simulink library "ebs_rebuild_generic_std"  (R2016a)
settings: Solver=VariableStepAuto  StartTime=0.0  StopTime=10.0  RelTol=1e-3
undefined symbols (not defined in the file): sMP
(part 1 of 2)
settings Model: Creator=CAB  LastModifiedBy=CAB
settings GRTTargetCC: GeneratePreprocessorConditionals=Use local settings

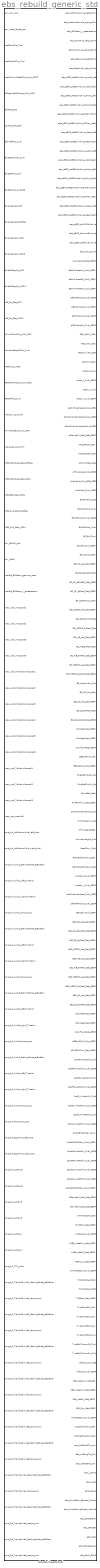
== system ebs_rebuild_generic_std ==
  ebs_rebuild_generic_std : Subsystem  mask{s1=sMP.ctrl.ebs.settings_iMode, s2=sMP.ctrl.ebs.settings_dt, initCmd='Parameters_ebs_rebuild_generic_std_sf', p1=sMP.ctrl.ebs.dim_xAxis_zSoll, p2=sMP.ctrl.ebs.veh.ABS_L1o, p3=sMP.ctrl.ebs.veh.ABS_L1v, p4=sMP.ctrl.ebs.veh.ABS_L2o, p5=sMP.ctrl.ebs.veh.ABS_L2v, p6=sMP.ctrl.ebs.veh.ABS_MinusB, p7=sMP.ctrl.ebs.veh.ABS_PlusB, p8=sMP.ctrl.ebs.veh.ABS_PlusOB, p9=sMP.ctrl.ebs.veh.ABS_THe, p10=sMP.ctrl.ebs.veh.ABS_TPulHold, p11=sMP.ctrl.ebs.veh.ABS_TPulOpen, p12=sMP.ctrl.ebs.veh.ABS_vMin_kmh, p13=sMP.ctrl.ebs.veh.flagTrailerABS, p14=sMP.ctrl.ebs.veh.rdynFA, p15=sMP.ctrl.ebs.veh.rdynRA, p16=sMP.ctrl.ebs.veh.rdynTA, p17=sMP.ctrl.ebs.veh.stepSize, p18=sMP.ctrl.ebs.ALB_dpMin_bar, p19=sMP.ctrl.ebs.ALB_mRA_Max_kg, p20=sMP.ctrl.ebs.ALB_mRA_Min_kg, p21=sMP.ctrl.ebs.ALB_p1Ref_bar, p22=sMP.ctrl.ebs.ALB_p2Max_bar, p23=sMP.ctrl.ebs.ALB_p2Min_bar, p24=sMP.ctrl.ebs.EBI_mueMax, p25=sMP.ctrl.ebs.EBI_vMin_kmh, p26=sMP.ctrl.ebs.flag_ABS, p27=sMP.ctrl.ebs.flag_DownhillDriveTest, p28=sMP.ctrl.ebs.flag_EBI, p29=sMP.ctrl.ebs.flag_SlopeCompActive, p30=sMP.ctrl.ebs.mec_iDiffAxle, p31=sMP.ctrl.ebs.Recuperation_end, p32=sMP.ctrl.ebs.Recuperation_initial, p33=sMP.ctrl.ebs.out.aAutoOpMd_Stat_SBSP, p34=sMP.ctrl.ebs.out.aBrkAirPressAA_Cval_SBSP, p35=sMP.ctrl.ebs.out.aBrkAirPressFA_Cval_SBSP, p36=sMP.ctrl.ebs.out.aBrkAirPressRA_Cval_SBSP, p37=sMP.ctrl.ebs.out.aBrkPdlPosn3_Cval_SBSP, p38=sMP.ctrl.ebs.out.aBrkTempFA_Cval_SBSP, p39=sMP.ctrl.ebs.out.aBrkTempIA_Cval_SBSP, p40=sMP.ctrl.ebs.out.aBrkTempRA_Cval_SBSP, p41=sMP.ctrl.ebs.out.ABS_Actv2_Stat, p42=sMP.ctrl.ebs.out.ABS_Actv_Stat, p43=sMP.ctrl.ebs.out.ABS_FullyOp_Stat, p44=sMP.ctrl.ebs.out.ABS_Trlr_Stat, p45=sMP.ctrl.ebs.out.Accel_X_Cval, p46=sMP.ctrl.ebs.out.Accel_X_Cval_SBSP, p47=sMP.ctrl.ebs.out.Accel_Y_Cval, p48=sMP.ctrl.ebs.out.Accel_Y_Cval_SBSP, p49=sMP.ctrl.ebs.in.ActlEmotTrq_Cval, p50=sMP.ctrl.ebs.in.ActlEngPctTrq_Cval, p51=sMP.ctrl.ebs.in.ActlMaxAvlRetPctTrq_Cval_CPC3, p52=sMP.ctrl.ebs.out.AddInfoVehSped_Cval_SBSP, p53=sMP.ctrl.ebs.out.aGroCmbVehWeight_Cval_SBSP, p54=sMP.ctrl.ebs.out.aGroCmbVehWeightConf_SBSP, p55=sMP.ctrl.ebs.in.aSbspVehBrkForce_Cmd_SDS, p56=sMP.ctrl.ebs.out.aStandstill_Dtct_Stat_SBSP, p57=sMP.ctrl.ebs.out.ATC_BrkCtrl_Stat, p58=sMP.ctrl.ebs.out.ATC_EngCtrl_Stat, p59=sMP.ctrl.ebs.out.ATC_InfoSgl_Stat, p60=sMP.ctrl.ebs.out.aTCV_Press_Cval_SBSP, p61=sMP.ctrl.ebs.out.aVehSpd_Cval_E2E_SBSP, p62=sMP.ctrl.ebs.out.aVehSpd_Cval_SBSP, p63=sMP.ctrl.ebs.out.BlockTend_Stat, p64=sMP.ctrl.ebs.out.BrkPdlPosn3_Cval, p65=sMP.ctrl.ebs.out.BrkPdlPosn3_Cval_SBSP, p66=sMP.ctrl.ebs.out.BrkPdlPosn_Cval, p67=sMP.ctrl.ebs.in.BrkPress_Rq, p68=sMP.ctrl.ebs.out.BS_Brk_Cval, p69=sMP.ctrl.ebs.out.BS_Brk_Cval_SBSP, p70=sMP.ctrl.ebs.out.BS_CS_Acc_Stat, p71=sMP.ctrl.ebs.out.BS_CS_Acc_Stat_SBSP, p72=sMP.ctrl.ebs.out.BS_CS_RqPerf2_Stat, p73=sMP.ctrl.ebs.out.BS_CS_RqPerf2_Stat_SBSP, p74=sMP.ctrl.ebs.out.BS_CS_RqPerf_Stat_SBSP, p75=sMP.ctrl.ebs.out.BS_CSCPC_Acc_Stat, p76=sMP.ctrl.ebs.out.BS_CSCPC_Acc_Stat_SBSP, p77=sMP.ctrl.ebs.out.BS_CSCPC_Intf_Stat, p78=sMP.ctrl.ebs.out.BS_CSCPC_RqPerf_Stat, p79=sMP.ctrl.ebs.out.BS_HB_Acc_Stat_SBSP, p80=sMP.ctrl.ebs.out.BS_HB_RqPerf_Stat, p81=sMP.ctrl.ebs.out.BS_HB_RqPerf_Stat_SBSP, p82=sMP.ctrl.ebs.out.BS_HBCPC_Acc_Stat_SBSP, p83=sMP.ctrl.ebs.out.BS_HBCPC_RqPerf_Stat_SBSP, p84=sMP.ctrl.ebs.out.BS_RoadIncln_Cval, p85=sMP.ctrl.ebs.out.BS_SS_Acc_Stat, p86=sMP.ctrl.ebs.out.BS_SS_Acc_Stat_SBSP, p87=sMP.ctrl.ebs.out.BS_SS_RqPerf_Stat, p88=sMP.ctrl.ebs.out.BS_SS_RqPerf_Stat_SBSP, p89=sMP.ctrl.ebs.in.Clutch_Stat_CPC, p90=sMP.ctrl.ebs.out.ConfLatAccel_SBSP, p91=sMP.ctrl.ebs.out.ConfLgtAccel_SBSP, p92=sMP.ctrl.ebs.out.ConfYawRate_SBSP, p93=sMP.ctrl.ebs.in.drv_BrkPdl_pos, p94=sMP.ctrl.ebs.in.drv_PkBrk, p95=sMP.ctrl.ebs.out.ebs_ActlEmotTrq_Nm, p96=sMP.ctrl.ebs.out.ebs_ActlEngTrq_Nm, p97=sMP.ctrl.ebs.out.ebs_ActlRetTrq_Nm, p98=sMP.ctrl.ebs.out.ebs_AdditionalAxle_left_pDmd, p99=sMP.ctrl.ebs.out.ebs_AdditionalAxle_right_pDmd, p100=sMP.ctrl.ebs.out.EBS_BrkSw2_Rq, p101=sMP.ctrl.ebs.out.EBS_BrkSw2_Rq_SBSP, p102=sMP.ctrl.ebs.out.ebs_ESCsens_y_acceleration, p103=sMP.ctrl.ebs.out.ebs_FrontAxle_left_pDmd, p104=sMP.ctrl.ebs.out.ebs_FrontAxle_right_pDmd, p105=sMP.ctrl.ebs.out.ebs_i_Emot, p106=sMP.ctrl.ebs.out.ebs_i_Ret, p107=sMP.ctrl.ebs.out.ebs_kappa, p108=sMP.ctrl.ebs.out.ebs_RearAxle_left_pDmd, p109=sMP.ctrl.ebs.out.ebs_RearAxle_right_pDmd, p110=sMP.ctrl.ebs.out.ebs_sBSP_stABSInValve_Addl_Left, p111=sMP.ctrl.ebs.out.ebs_sBSP_stABSInValve_Addl_Right, p112=sMP.ctrl.ebs.out.ebs_sBSP_stABSInValve_Front_Left, p113=sMP.ctrl.ebs.out.ebs_sBSP_stABSInValve_Front_Right, p114=sMP.ctrl.ebs.out.ebs_sBSP_stABSInValve_RCMax_Front, p115=sMP.ctrl.ebs.out.ebs_sBSP_stABSInValve_RCMax_Rear, p116=sMP.ctrl.ebs.out.ebs_sBSP_stABSInValve_Rear_Left, p117=sMP.ctrl.ebs.out.ebs_sBSP_stABSInValve_Rear_Right, p118=sMP.ctrl.ebs.out.ebs_sBSP_stABSOutValve_Addl_Left, p119=sMP.ctrl.ebs.out.ebs_sBSP_stABSOutValve_Addl_Right, p120=sMP.ctrl.ebs.out.ebs_sBSP_stABSOutValve_Front_Left, p121=sMP.ctrl.ebs.out.ebs_sBSP_stABSOutValve_Front_Right, p122=sMP.ctrl.ebs.out.ebs_sBSP_stABSOutValve_RCMax_Front, p123=sMP.ctrl.ebs.out.ebs_sBSP_stABSOutValve_RCMax_Rear, p124=sMP.ctrl.ebs.out.ebs_sBSP_stABSOutValve_Rear_Left, p125=sMP.ctrl.ebs.out.ebs_sBSP_stABSOutValve_Rear_Right, p126=sMP.ctrl.ebs.out.ebs_sBSP_stAPCVBuValve, p127=sMP.ctrl.ebs.out.ebs_sBSP_stAxmoBuValve, p128=sMP.ctrl.ebs.out.ebs_sBSP_stCMaxBuValve, p129=sMP.ctrl.ebs.out.ebs_SumBrakingForces_Trailer, p130=sMP.ctrl.ebs.out.ebs_SumBrakingForces_Vehicle, p131=sMP.ctrl.ebs.out.ebs_TCV_pDmd, p132=sMP.ctrl.ebs.out.ebs_zReqBrake, p133=sMP.ctrl.ebs.out.ebs_zReqEB, p134=sMP.ctrl.ebs.out.ebs_zRet, p135=sMP.ctrl.ebs.out.ebs_zSlopeComp, p136=sMP.ctrl.ebs.out.ebs_zSoll_BWG, p137=sMP.ctrl.ebs.in.EdrvRefTrq_Cval, p138=sMP.ctrl.ebs.in.EngPctTrqActl_Cval, p139=sMP.ctrl.ebs.in.EngRefTrq_Cval, p140=sMP.ctrl.ebs.out.EngRetTrqMax_Rq, p141=sMP.ctrl.ebs.out.EngRetTrqMin_Rq, p142=sMP.ctrl.ebs.in.EngRPM_Cval_CPC3, p143=sMP.ctrl.ebs.in.env_curv_pm, p144=sMP.ctrl.ebs.in.env_road_slope_pct, p145=sMP.ctrl.ebs.in.ExtAccel_Rq_CPC5ce, p146=sMP.ctrl.ebs.in.ExtAccel_Rq_CPC, p147=sMP.ctrl.ebs.in.ExtAccel_Rq_VRDU3, p148=sMP.ctrl.ebs.in.ExtAccel_Rq_VRDU, p149=sMP.ctrl.ebs.in.ExtBrkStat_Rq_CPC, p150=sMP.ctrl.ebs.in.ExtBrkStat_Rq_VRDU, p151=sMP.ctrl.ebs.out.FoundBrk_Stat, p152=sMP.ctrl.ebs.out.FullBrkAllow_Stat_SBSP, p153=sMP.ctrl.ebs.out.GroCmbVehWeight_Cval, p154=sMP.ctrl.ebs.in.HB_Rq_Stat_CPC, p155=sMP.ctrl.ebs.in.HB_Rq_Stat_VRDU, p156=sMP.ctrl.ebs.out.HillHolderAvl_Stat, p157=sMP.ctrl.ebs.in.mec3d_ESCsens_gamma_rate, p158=sMP.ctrl.ebs.in.mec3d_ESCsens_y_acceleration, p159=sMP.ctrl.ebs.in.mec_veh_AxleLoad1, p160=sMP.ctrl.ebs.in.mec_veh_AxleLoad2, p161=sMP.ctrl.ebs.in.mec_veh_AxleLoad3, p162=sMP.ctrl.ebs.in.mec_veh_AxleLoad4, p163=sMP.ctrl.ebs.in.mec_veh_Trailer02AxleLoad1, p164=sMP.ctrl.ebs.in.mec_veh_Trailer02AxleLoad2, p165=sMP.ctrl.ebs.in.mec_veh_Trailer02AxleLoad3, p166=sMP.ctrl.ebs.in.mec_veh_Trailer02AxleLoad4, p167=sMP.ctrl.ebs.in.mec_veh_Trailer02AxleLoad5, p168=sMP.ctrl.ebs.in.mec_veh_Trailer02AxleLoad6, p169=sMP.ctrl.ebs.in.mec_veh_TrailerAxleLoad1, p170=sMP.ctrl.ebs.in.mec_veh_TrailerAxleLoad2, p171=sMP.ctrl.ebs.in.mec_veh_TrailerAxleLoad3, p172=sMP.ctrl.ebs.in.mec_veh_transVel, p173=sMP.ctrl.ebs.in.MinAvlEmotTrq_Cval_CPC, p174=sMP.ctrl.ebs.in.NomFrictEngPctTrq_Cval, p175=sMP.ctrl.ebs.out.NrTrlr_Stat_SBSP, p176=sMP.ctrl.ebs.in.PkBrk_Rq_VRDU, p177=sMP.ctrl.ebs.in.pne_brk_AdditionalAxle_left_pAct, p178=sMP.ctrl.ebs.in.pne_brk_AdditionalAxle_right_pAct, p179=sMP.ctrl.ebs.in.pne_brk_Axle1_BrakingForce_at8p5bar, p180=sMP.ctrl.ebs.in.pne_brk_Axle1_left_Tinterior, p181=sMP.ctrl.ebs.in.pne_brk_Axle1_right_Tinterior, p182=sMP.ctrl.ebs.in.pne_brk_Axle1_torque_sns, p183=sMP.ctrl.ebs.in.pne_brk_Axle2_BrakingForce_at8p5bar, p184=sMP.ctrl.ebs.in.pne_brk_Axle2_left_Tinterior, p185=sMP.ctrl.ebs.in.pne_brk_Axle2_right_Tinterior, p186=sMP.ctrl.ebs.in.pne_brk_Axle2_torque_sns, p187=sMP.ctrl.ebs.in.pne_brk_Axle3_BrakingForce_at8p5bar, p188=sMP.ctrl.ebs.in.pne_brk_Axle3_left_Tinterior, p189=sMP.ctrl.ebs.in.pne_brk_Axle3_right_Tinterior, p190=sMP.ctrl.ebs.in.pne_brk_Axle3_torque_sns, p191=sMP.ctrl.ebs.in.pne_brk_Axle4_BrakingForce_at8p5bar, p192=sMP.ctrl.ebs.in.pne_brk_Axle4_left_Tinterior, p193=sMP.ctrl.ebs.in.pne_brk_Axle4_right_Tinterior, p194=sMP.ctrl.ebs.in.pne_brk_Axle4_torque_sns, p195=sMP.ctrl.ebs.in.pne_brk_FrontAxle_pAct, p196=sMP.ctrl.ebs.in.pne_brk_RearAxle_left_pAct, p197=sMP.ctrl.ebs.in.pne_brk_RearAxle_right_pAct, p198=sMP.ctrl.ebs.in.pne_brk_rotVel_al, p199=sMP.ctrl.ebs.in.pne_brk_rotVel_ar, p200=sMP.ctrl.ebs.in.pne_brk_rotVel_fl, p201=sMP.ctrl.ebs.in.pne_brk_rotVel_fr, p202=sMP.ctrl.ebs.in.pne_brk_rotVel_rl, p203=sMP.ctrl.ebs.in.pne_brk_rotVel_rr, p204=sMP.ctrl.ebs.in.pne_brk_TCV_pAct, p205=sMP.ctrl.ebs.in.pne_brk_Trailer02Axle1_BrakingForce_at8p5bar, p206=sMP.ctrl.ebs.in.pne_brk_Trailer02Axle1_torque_sns, p207=sMP.ctrl.ebs.in.pne_brk_Trailer02Axle2_BrakingForce_at8p5bar, p208=sMP.ctrl.ebs.in.pne_brk_Trailer02Axle2_torque_sns, p209=sMP.ctrl.ebs.in.pne_brk_Trailer02Axle3_BrakingForce_at8p5bar, p210=sMP.ctrl.ebs.in.pne_brk_Trailer02Axle3_torque_sns, p211=sMP.ctrl.ebs.in.pne_brk_Trailer02Axle4_BrakingForce_at8p5bar, p212=sMP.ctrl.ebs.in.pne_brk_Trailer02Axle4_torque_sns, p213=sMP.ctrl.ebs.in.pne_brk_Trailer02Axle5_BrakingForce_at8p5bar, p214=sMP.ctrl.ebs.in.pne_brk_Trailer02Axle5_torque_sns, p215=sMP.ctrl.ebs.in.pne_brk_Trailer02Axle6_BrakingForce_at8p5bar, p216=sMP.ctrl.ebs.in.pne_brk_Trailer02Axle6_torque_sns, p217=sMP.ctrl.ebs.in.pne_brk_TrailerAxle1_BrakingForce_at8p5bar, p218=sMP.ctrl.ebs.in.pne_brk_TrailerAxle1_torque_sns, p219=sMP.ctrl.ebs.in.pne_brk_TrailerAxle2_BrakingForce_at8p5bar, p220=sMP.ctrl.ebs.in.pne_brk_TrailerAxle2_torque_sns, p221=sMP.ctrl.ebs.in.pne_brk_TrailerAxle3_BrakingForce_at8p5bar, p222=sMP.ctrl.ebs.in.pne_brk_TrailerAxle3_torque_sns, p223=sMP.ctrl.ebs.out.PwrVehWeight_Cval, p224=sMP.ctrl.ebs.in.RetPctTrqActl2_Cval_CPC3, p225=sMP.ctrl.ebs.in.RetRefTrq_Cval, p226=sMP.ctrl.ebs.out.RoadCurv_Cval, p227=sMP.ctrl.ebs.out.ROP_BrkCtrlActv2_Stat, p228=sMP.ctrl.ebs.out.ROP_EngCtrlActv2_Stat, p229=sMP.ctrl.ebs.out.sAccel_X_Cval_SBSP, p230=sMP.ctrl.ebs.out.sAccel_Y_Cval_SBSP, p231=sMP.ctrl.ebs.out.sAddInfoVehSped_Cval_SBSP, p232=sMP.ctrl.ebs.out.sBrkPdlPosn3_Cval_SBSP, p233=sMP.ctrl.ebs.out.sBS_Brk_Cval_SBSP, p234=sMP.ctrl.ebs.out.sBS_CS_Acc_Stat_SBSP, p235=sMP.ctrl.ebs.out.sBS_CS_RqPerf2_Stat_SBSP, p236=sMP.ctrl.ebs.out.sBS_CS_RqPerf_Stat_SBSP, p237=sMP.ctrl.ebs.out.sBS_CSCPC_Acc_Stat_SBSP, p238=sMP.ctrl.ebs.out.sBS_HB_Acc_Stat_SBSP, p239=sMP.ctrl.ebs.out.sBS_HB_RqPerf_Stat_SBSP, p240=sMP.ctrl.ebs.out.sBS_HBCPC_Acc_Stat_SBSP, p241=sMP.ctrl.ebs.out.sBS_HBCPC_RqPerf_Stat_SBSP, p242=sMP.ctrl.ebs.out.sBS_SS_Acc_Stat_SBSP, p243=sMP.ctrl.ebs.out.sBS_SS_RqPerf_Stat_SBSP, p244=sMP.ctrl.ebs.out.sConfLatAccel_SBSP, p245=sMP.ctrl.ebs.out.sConfLgtAccel_SBSP, p246=sMP.ctrl.ebs.out.sConfYawRate_SBSP, p247=sMP.ctrl.ebs.out.sEBS_BrkSw2_Rq_SBSP, p248=sMP.ctrl.ebs.out.sFullBrkAllow_Stat_SBSP, p249=sMP.ctrl.ebs.out.SpdFtAxleLtWhl_Cval, p250=sMP.ctrl.ebs.out.SpdFtAxleLtWhl_Cval_SBSP, p251=sMP.ctrl.ebs.out.SpdFtAxleRtWhl_Cval, p252=sMP.ctrl.ebs.out.SpdFtAxleRtWhl_Cval_SBSP, p253=sMP.ctrl.ebs.out.SpdR_AxleLtWhl_Cval, p254=sMP.ctrl.ebs.out.SpdR_AxleLtWhl_Cval_SBSP, p255=sMP.ctrl.ebs.out.SpdR_AxleRtWhl_Cval, p256=sMP.ctrl.ebs.out.SpdR_AxleRtWhl_Cval_SBSP, p257=sMP.ctrl.ebs.out.SrcAdrBrkCtrlDev_Cval, p258=sMP.ctrl.ebs.out.SrcAdrBrkCtrlDev_Cval_SBSP, p259=sMP.ctrl.ebs.out.sSpdFtAxleLtWhl_Cval_SBSP, p260=sMP.ctrl.ebs.out.sSpdFtAxleRtWhl_Cval_SBSP, p261=sMP.ctrl.ebs.out.sSpdR_AxleLtWhl_Cval_SBSP, p262=sMP.ctrl.ebs.out.sSpdR_AxleRtWhl_Cval_SBSP, p263=sMP.ctrl.ebs.out.sSrcAdrBrkCtrlDev_Cval_SBSP, p264=sMP.ctrl.ebs.out.sStandstill_Dtct_Stat_SBSP, p265=sMP.ctrl.ebs.out.Standstill_Dtct_Stat_SBSP, p266=sMP.ctrl.ebs.out.sTrlrAbsOper_Stat, p267=sMP.ctrl.ebs.out.sTrlrEstm_Stat_SBSP, p268=sMP.ctrl.ebs.out.sVehSpd_Cval_SBSP, p269=sMP.ctrl.ebs.out.sXBR_AccelLim_Stat_SBSP, p270=sMP.ctrl.ebs.out.sXBR_ActCtrl_Stat_SBSP, p271=sMP.ctrl.ebs.out.sXBR_Sys_Stat_SBSP, p272=sMP.ctrl.ebs.out.sYawRateCorr_Cval_SBSP, p273=sMP.ctrl.ebs.out.TrctrAbsOper_Stat, p274=sMP.ctrl.ebs.out.TrlrAbsOper_Stat, p275=sMP.ctrl.ebs.out.TrlrEstm_Stat_SBSP, p276=sMP.ctrl.ebs.in.TrqConv_Cval_PT, p277=sMP.ctrl.ebs.in.TxInShaftSpd_Cval_CPC, p278=sMP.ctrl.ebs.out.TyreCorrLtFA_Cval, p279=sMP.ctrl.ebs.out.TyreCorrLtRA_Cval, p280=sMP.ctrl.ebs.out.TyreCorrRtFA_Cval, p281=sMP.ctrl.ebs.out.TyreCorrRtRA_Cval, p282=sMP.ctrl.ebs.out.TyreRollCircumFA_Cval, p283=sMP.ctrl.ebs.out.TyreRollCircumRA_Cval, p284=sMP.ctrl.ebs.in.VehSpd1_Cval_Trlr, p285=sMP.ctrl.ebs.out.VehSpd_Cval_BS, p286=sMP.ctrl.ebs.out.VehSpd_Cval_SBSP, p287=sMP.ctrl.ebs.out.XBR_AccelLim_Stat_BS, p288=sMP.ctrl.ebs.out.XBR_AccelLim_Stat_SBSP, p289=sMP.ctrl.ebs.out.XBR_ActCtrl_Stat_SBSP, p290=sMP.ctrl.ebs.in.XBR_CtrlMode_Stat_CPC5ce, p291=sMP.ctrl.ebs.in.XBR_CtrlMode_Stat_VRDU, p292=sMP.ctrl.ebs.in.XBR_EBI_Stat_VRDU, p293=sMP.ctrl.ebs.in.XBR_Prio_Stat_CPC5ce, p294=sMP.ctrl.ebs.in.XBR_Prio_Stat_VRDU, p295=sMP.ctrl.ebs.out.XBR_Sys_Stat_SBSP, p296=sMP.ctrl.ebs.out.YawRateCorr_Cval_SBSP, p297=sMP.ctrl.ebs.out.YC_BrkCtrlActv2_Stat, p298=sMP.ctrl.ebs.out.YC_EngCtrlActv2_Stat, p299=sMP.ctrl.ebs.zSoll_dx_xAxis_nom, p300=sMP.ctrl.ebs.zSoll_dx_yAxis_nom, p301=sMP.ctrl.ebs.veh.axleLoadTrailer02_kg, p302=sMP.ctrl.ebs.veh.axleLoadTrailer_kg, p303=sMP.ctrl.ebs.veh.axleLoadVehicle_kg, p304=sMP.ctrl.ebs.veh.brkCircuit, p305=sMP.ctrl.ebs.veh.flagTrailer02ControlActive, p306=sMP.ctrl.ebs.veh.flagTrailerControlActive, p307=sMP.ctrl.ebs.veh.pAppCyl_Tractor, p308=sMP.ctrl.ebs.veh.pAppCyl_Trailer, p309=sMP.ctrl.ebs.veh.pAppCyl_Trailer02, p310=sMP.ctrl.ebs.veh.rdynTrailer02, p311=sMP.ctrl.ebs.veh.speedSensorPosnVeh}
      mask prompts: s1 "Solver Type: settings_iMode [-]"; s2 "Solver Step Size: settings_dt [s]"; initCmd "Initialization command"; p1 "Dimension x-Axis zSoll-Curve [max. 40] export=true name=dim_xAxis_zSoll prio=1 dataSetName=ebs_dummy dataClassType=main dataClassName=main  unit='-' description='Dimension x-Axis zSoll-Curve': BWG.dim_xAxis_zSoll [-]"; p2 "Velocity Offset L1o (km/h) export=true name=ABS_L1o prio=1 dataSetName=veh_dummy dataClassType=veh dataClassName=veh unit='km/h' description='Velocity Offset L1o (km/h)': eBS_veh_Param.ABS_L1o [-]"; p3 "Speed Fraction for Threshold Speed 1 (0.01%) export=true name=ABS_L1v prio=1 dataSetName=veh_dummy dataClassType=veh dataClassName=veh unit='' description='Speed Fraction for Threshold Speed 1 (0.01%)': eBS_veh_Param.ABS_L1v [-]"; p4 "Velocity Offset L2o (km/h) export=true name=ABS_L2o prio=1 dataSetName=veh_dummy dataClassType=veh dataClassName=veh unit='km/h' description='Velocity Offset L2o (km/h)': eBS_veh_Param.ABS_L2o [-]"; p5 "Speed Fraction for Threshold Speed 2 (0.01%) export=true name=ABS_L2v prio=1 dataSetName=veh_dummy dataClassType=veh dataClassName=veh unit='' description='Speed Fraction for Threshold Speed 2 (0.01%)': eBS_veh_Param.ABS_L2v [-]"; p6 "Decceleration Threshold in [g] export=true name=ABS_MinusB prio=1 dataSetName=veh_dummy dataClassType=veh dataClassName=veh unit='' description='Decceleration Threshold in [g]': eBS_veh_Param.ABS_MinusB [-]"; p7 "Acceleration Threshold in [g] export=true name=ABS_PlusB prio=1 dataSetName=veh_dummy dataClassType=veh dataClassName=veh unit='' description='Decceleration Threshold in [g]': eBS_veh_Param.ABS_PlusB [-]"; p8 "Upper Acceleration Threshold in [g] export=true name=ABS_PlusOB prio=1 dataSetName=veh_dummy dataClassType=veh dataClassName=veh unit='' description='Upper Acceleration Threshold in [g]': eBS_veh_Param.ABS_PlusOB [-]"; p9 "Holding Time [ms] export=true name=ABS_THe prio=1 dataSetName=veh_dummy dataClassType=veh dataClassName=veh unit='ms' description='Holding Time [ms]': eBS_veh_Param.ABS_THe [-]"; p10 "Holding Time for Pulsating Pressure Build-Up [ms] export=true name=ABS_TPulHold prio=1 dataSetName=veh_dummy dataClassType=veh dataClassName=veh unit='ms' description='Holding Time for Pulsating Pressure Build-Up [ms]': eBS_veh_Param.ABS_TPulHold [-]"; p11 "Opening Time for Pulsating Pressure Build-Up [ms] export=true name=ABS_TPulOpen prio=1 dataSetName=veh_dummy dataClassType=veh dataClassName=veh unit='ms' description='Opening Time for Pulsating Pressure Build-Up [ms]': eBS_veh_Param.ABS_TPulOpen [-]"; p12 "Minimum Velocity for ABS Activity [km/h] export=true name=ABS_vMin_kmh prio=1 dataSetName=veh_dummy dataClassType=veh dataClassName=veh unit='km/h' description='Minimum Velocity for ABS Activity [km/h]': eBS_veh_Param.ABS_vMin_kmh [-]"; p13 "Trailer ABS Config (0 - none, 1- ABS, 2 - EBS (incl. ABS)), used in pneAux export=true name=flagTrailerABS prio=1 dataSetName=veh_dummy dataClassType=veh dataClassName=veh unit='-' description='Trailer ABS Config (0 - none, 1- ABS, 2 - EBS (incl. ABS))': eBS_veh_Param.flagTrailerABS [-]"; p14 "Dyn. Wheel Radius Front Axle [mm] export=true name=rdynFA prio=1 dataSetName=veh_dummy dataClassType=veh dataClassName=veh unit='mm' description='Dyn. Wheel Radius Front Axle [mm]': eBS_veh_Param.rdynFA [-]"; p15 "Dyn. Wheel Radius Rear Axle [mm] export=true name=rdynRA prio=1 dataSetName=veh_dummy dataClassType=veh dataClassName=veh unit='mm' description='Dyn. Wheel Radius Rear Axle [mm]': eBS_veh_Param.rdynRA [-]"; p16 "Dyn. Wheel Radius Trailer Axle [mm] export=true name=rdynTA prio=1 dataSetName=veh_dummy dataClassType=veh dataClassName=veh unit='mm' description='Dyn. Wheel Radius Trailer Axle [mm]': eBS_veh_Param.rdynTA [-]"; p17 "step Size [s] export=true name=stepSize prio=1 dataSetName=veh_dummy dataClassType=veh dataClassName=veh unit='s' description=' step size [s]': eBS_veh_Param.stepSize [s]"; p18 "ALB Linear Pressure Range p2/p1->1:1 export=true name=ALB_dpMin_bar prio=1 dataSetName=ebs_dummy dataClassType=main dataClassName=main unit=bar description='ALB Linear Pressure Range p2/p1->1:1': eBSParam.ALB_dpMin_bar [-]"; p19 "ALB Maximal Rear Axle Load for p2Max [kg] export=true name=ALB_mRA_Max_kg prio=1 dataSetName=ebs_dummy dataClassType=main dataClassName=main unit=kg description='ALB Maximal Rear Axle Load for p2Max [kg]': eBSParam.ALB_mRA_Max_kg [-]"; p20 "ALB Minimal Rear Axle Load for p2Min [kg] export=true name=ALB_mRA_Min_kg prio=1 dataSetName=ebs_dummy dataClassType=main dataClassName=main unit=kg description='ALB Minimal Rear Axle Load for p2Min [kg]': eBSParam.ALB_mRA_Min_kg [-]"; p21 "ALB Reference Inlet Pressure p1 [bar] export=true name=ALB_p1Ref_bar prio=1 dataSetName=ebs_dummy dataClassType=main dataClassName=main unit=bar description='ALB Reference Inlet Pressure p1 [bar]': eBSParam.ALB_p1Ref_bar [-]"; p22 "ALB Maximum Pressure at mRA_Max_kg [bar] export=true name=ALB_p2Max_bar prio=1 dataSetName=ebs_dummy dataClassType=main dataClassName=main unit=bar description='ALB Maximum Pressure at mRA_Max_kg [bar]': eBSParam.ALB_p2Max_bar [-]"; p23 "ALB Minimum Pressure at mRA_Min [bar] export=true name=ALB_p2Min_bar prio=1 dataSetName=ebs_dummy dataClassType=main dataClassName=main unit=bar description='ALB Minimum Pressure at mRA_Min [bar]': eBSParam.ALB_p2Min_bar [-]"; p24 "Maximum Friction Coefficient Rear Axle export=true name=EBI_mueMax prio=1 dataSetName=ebs_dummy dataClassType=main dataClassName=main unit='-' description='Maximum Friction Coefficient Rear Axle': eBSParam.EBI_mueMax [-]"; p25 "Minum Initial Velocity [km/h] (eBIActive>EBI_vMin_kmh) export=true name=EBI_vMin_kmh prio=1 dataSetName=ebs_dummy dataClassType=main dataClassName=main unit='km/h' description='Minum Initial Velocity [km/h] (eBIActive>EBI_vMin_kmh)': eBSParam.EBI_vMin_kmh [-]"; p26 "Vehicle with ABS-Brake System [0-false,1-true] export=true name=flag_ABS prio=1 dataSetName=ebs_dummy dataClassType=main dataClassName=main unit='-' description='Vehicle with ABS-Brake System [0-false,1-true]': eBSParam.flag_ABS [-]"; p27 "Flag Downhill Drive Test [0-false,1-true] export=true name=flag_DownhillDriveTest prio=1 dataSetName=ebs_dummy dataClassType=main dataClassName=main unit='-' description='Flag Downhill Drive Test [0-false,1-true]': eBSParam.flag_DownhillDriveTest [-]"; p28 "Endurance Brake Integration (EBI) [0-no EBI,1-EBI, base deceleration of 2% by service brake, 2- EBI 100%, 3 - prior endurance brake activation, 4 - EBI Bus mode] export=true name=flag_EBI prio=1 dataSetName=ebs_dummy dataClassType=main dataClassName=main unit='-' description='Endurance Brake Integration (EBI) [0-no EBI,1-EBI, base deceleration of 2% by service brake, 2- EBI 100%, 3 - prior endurance brake activation, 4 - EBI Bus mode]': eBSParam.flag_EBI [-]"; p29 "Slope Compensation Active [0 - false,1 - true] export=true name=flag_SlopeCompActive prio=1 dataSetName=ebs_dummy dataClassType=main dataClassName=main unit='-' description='Slope Compensation Active [0 - false,1 - true]': eBSParam.flag_SlopeCompActive [-]"; p30 "Transmission Ratio EMot - Axle [-] export=true name=mec_iDiffAxle prio=1 dataSetName=ebs_dummy dataClassType=main dataClassName=main unit='' description='Transmission Ratio EMot - Axle [-]': eBSParam.mec_iDiffAxle [-]"; p31 "Recuperation value for full brake pedal actuation [Nm] export=true name=Recuperation_end prio=1 dataSetName=ebs_dummy dataClassType=main dataClassName=main unit=kg description='Recuperation value for inital brake pedal actuation [Nm] ': eBSParam.Recuperation_end [-]"; p32 "Recuperation value for inital brake pedal actuation [Nm] export=true name=Recuperation_initial prio=1 dataSetName=ebs_dummy dataClassType=main dataClassName=main unit=kg description='Recuperation value for inital brake pedal actuation [Nm] ': eBSParam.Recuperation_initial [-]"; p33 "aAutoOpMd_Stat_SBSP export=true name=aAutoOpMd_Stat_SBSP prio=1 dataSetName=std dataClassType=initIO dataClassName=initIO unit='-' description='aAutoOpMd_Stat_SBSP': IO_EBS_InputSignals.aAutoOpMd_Stat_SBSP_0 [-]"; p34 "aBrkAirPressAA_Cval_SBSP export=true name=aBrkAirPressAA_Cval_SBSP prio=1 dataSetName=std dataClassType=initIO dataClassName=initIO unit='kPa' description='aBrkAirPressAA_Cval_SBSP': IO_EBS_InputSignals.aBrkAirPressAA_Cval_SBSP_0 [-]"; p35 "aBrkAirPressFA_Cval_SBSP export=true name=aBrkAirPressFA_Cval_SBSP prio=1 dataSetName=std dataClassType=initIO dataClassName=initIO unit='kPa' description='aBrkAirPressFA_Cval_SBSP': IO_EBS_InputSignals.aBrkAirPressFA_Cval_SBSP_0 [-]"; p36 "aBrkAirPressRA_Cval_SBSP export=true name=aBrkAirPressRA_Cval_SBSP prio=1 dataSetName=std dataClassType=initIO dataClassName=initIO unit='kPa' description='aBrkAirPressRA_Cval_SBSP': IO_EBS_InputSignals.aBrkAirPressRA_Cval_SBSP_0 [-]"; p37 "aBrkPdlPosn3_Cval_SBSP export=true name=aBrkPdlPosn3_Cval_SBSP prio=1 dataSetName=std dataClassType=initIO dataClassName=initIO unit='%' description='aBrkPdlPosn3_Cval_SBSP': IO_EBS_InputSignals.aBrkPdlPosn3_Cval_SBSP_0 [-]"; p38 "aBrkTempFA_Cval_SBSP export=true name=aBrkTempFA_Cval_SBSP prio=1 dataSetName=std dataClassType=initIO dataClassName=initIO unit='degC' description='aBrkTempFA_Cval_SBSP': IO_EBS_InputSignals.aBrkTempFA_Cval_SBSP_0 [-]"; p39 "aBrkTempIA_Cval_SBSP export=true name=aBrkTempIA_Cval_SBSP prio=1 dataSetName=std dataClassType=initIO dataClassName=initIO unit='degC' description='aBrkTempIA_Cval_SBSP': IO_EBS_InputSignals.aBrkTempIA_Cval_SBSP_0 [-]"; p40 "aBrkTempRA_Cval_SBSP export=true name=aBrkTempRA_Cval_SBSP prio=1 dataSetName=std dataClassType=initIO dataClassName=initIO unit='degC' description='aBrkTempRA_Cval_SBSP': IO_EBS_InputSignals.aBrkTempRA_Cval_SBSP_0 [-]"; p41 "ABS_Actv2_Stat export=true name=ABS_Actv2_Stat prio=1 dataSetName=std dataClassType=initIO dataClassName=initIO unit='-' description='ABS_Actv2_Stat': IO_EBS_InputSignals.ABS_Actv2_Stat_0 [-]"; p42 "ABS_Actv_Stat export=true name=ABS_Actv_Stat prio=1 dataSetName=std dataClassType=initIO dataClassName=initIO unit='-' description='ABS_Actv_Stat': IO_EBS_InputSignals.ABS_Actv_Stat_0 [-]"; p43 "ABS_FullyOp_Stat export=true name=ABS_FullyOp_Stat prio=1 dataSetName=std dataClassType=initIO dataClassName=initIO unit='-' description='ABS_FullyOp_Stat': IO_EBS_InputSignals.ABS_FullyOp_Stat_0 [-]"; p44 "ABS_Trlr_Stat export=true name=ABS_Trlr_Stat prio=1 dataSetName=std dataClassType=initIO dataClassName=initIO unit='-' description='ABS_Trlr_Stat': IO_EBS_InputSignals.ABS_Trlr_Stat_0 [-]"; p45 "ABS61449S_E_LongitudAcc, 255 SNA; export=true name=Accel_X_Cval prio=1 dataSetName=std dataClassType=initIO dataClassName=initIO unit='m/s^2' description='ABS61449S_E_LongitudAcc, 255 SNA;': IO_EBS_InputSignals.Accel_X_Cval_0 [-]"; p46 "ABS61449S_E_LongitudAcc, 255 SNA; export=true name=Accel_X_Cval_SBSP prio=1 dataSetName=std dataClassType=initIO dataClassName=initIO unit='m/s^2' description='ABS61449S_E_LongitudAcc, 255 SNA;': IO_EBS_InputSignals.Accel_X_Cval_SBSP_0 [-]"; p47 "Accel_Y_Cval export=true name=Accel_Y_Cval prio=1 dataSetName=std dataClassType=initIO dataClassName=initIO unit=m/s^2 description='Accel_Y_Cval': IO_EBS_InputSignals.Accel_Y_Cval_0 [-]"; p48 "Accel_Y_Cval_SBSP export=true name=Accel_Y_Cval_SBSP prio=1 dataSetName=std dataClassType=initIO dataClassName=initIO unit=m/s^2 description='Accel_Y_Cval_SBSP': IO_EBS_InputSignals.Accel_Y_Cval_SBSP_0 [-]"; p49 "ActlEmotTrq_Cval (init) export=true name=ActlEmotTrq_Cval prio=1 dataSetName=std dataClassType=initIO dataClassName=initIO unit='-' description='ActlEmotTrq_Cval (init)': IO_EBS_InputSignals.ActlEmotTrq_Cval_0 [-]"; p50 "ActlEngPctTrq_Cval export=true name=ActlEngPctTrq_Cval prio=1 dataSetName=std dataClassType=initIO dataClassName=initIO unit='-' description='ActlEngPctTrq_Cval': IO_EBS_InputSignals.ActlEngPctTrq_Cval_0 [-]"; p51 "ActlMaxAvlRetPctTrq_Cval_CPC3 export=true name=ActlMaxAvlRetPctTrq_Cval_CPC3 prio=1 dataSetName=std dataClassType=initIO dataClassName=initIO unit='-' description='ActlMaxAvlRetPctTrq_Cval_CPC3': IO_EBS_InputSignals.ActlMaxAvlRetPctTrq_Cval_CPC3_0 [-]"; p52 "AddInfoVehSped_Cval_SBSP (init) export=true name=AddInfoVehSped_Cval_SBSP prio=1 dataSetName=std dataClassType=initIO dataClassName=initIO unit='' description='AddInfoVehSped_Cval_SBSP': IO_EBS_InputSignals.AddInfoVehSped_Cval_SBSP_0 [-]"; p53 "aGroCmbVehWeight_Cval_SBSP export=true name=aGroCmbVehWeight_Cval_SBSP prio=1 dataSetName=std dataClassType=initIO dataClassName=initIO unit='kg' description='aGroCmbVehWeight_Cval_SBSP': IO_EBS_InputSignals.aGroCmbVehWeight_Cval_SBSP_0 [-]"; p54 "aGroCmbVehWeightConf_SBSP export=true name=aGroCmbVehWeightConf_SBSP prio=1 dataSetName=std dataClassType=initIO dataClassName=initIO unit='%' description='Vehicle Mass estimate confidence factor': IO_EBS_InputSignals.aGroCmbVehWeightConf_SBSP_0 [-]"; p55 "aSbspVehBrkForce_Cmd_SDS export=true name=aSbspVehBrkForce_Cmd_SDS prio=1 dataSetName=std dataClassType=initIO dataClassName=initIO unit='N' description='aSbspVehBrkForce_Cmd_SDS': IO_EBS_InputSignals.aSbspVehBrkForce_Cmd_SDS_0 [-]"; p56 "aStandstill_Dtct_Stat_SBSP export=true name=aStandstill_Dtct_Stat_SBSP prio=1 dataSetName=std dataClassType=initIO dataClassName=initIO unit='-' description='Standstill detected Current state': IO_EBS_InputSignals.aStandstill_Dtct_Stat_SBSP_0 [-]"; p57 "ATC_BrkCtrl_Stat export=true name=ATC_BrkCtrl_Stat prio=1 dataSetName=std dataClassType=initIO dataClassName=initIO unit='-' description='ATC_BrkCtrl_Stat': IO_EBS_InputSignals.ATC_BrkCtrl_Stat_0 [-]"; p58 "ATC_EngCtrl_Stat export=true name=ATC_EngCtrl_Stat prio=1 dataSetName=std dataClassType=initIO dataClassName=initIO unit='-' description='ATC_EngCtrl_Stat': IO_EBS_InputSignals.ATC_EngCtrl_Stat_0 [-]"; p59 "ATC_InfoSgl_Stat export=true name=ATC_InfoSgl_Stat prio=1 dataSetName=std dataClassType=initIO dataClassName=initIO unit='-' description='ATC_InfoSgl_Stat': IO_EBS_InputSignals.ATC_InfoSgl_Stat_0 [-]"; p60 "aTCV_Press_Cval_SBSP export=true name=aTCV_Press_Cval_SBSP prio=1 dataSetName=std dataClassType=initIO dataClassName=initIO unit='kPa' description='aTCV_Press_Cval_SBSP': IO_EBS_InputSignals.aTCV_Press_Cval_SBSP_0 [-]"; p61 "aVehSpd_Cval_E2E_SBSP export=true name=aVehSpd_Cval_E2E_SBSP prio=1 dataSetName=std dataClassType=initIO dataClassName=initIO unit='km/h' description='aVehSpd_Cval_E2E_SBSP': IO_EBS_InputSignals.aVehSpd_Cval_E2E_SBSP_0 [-]"; p62 "aVehSpd_Cval_SBSP export=true name=aVehSpd_Cval_SBSP prio=1 dataSetName=std dataClassType=initIO dataClassName=initIO unit='km/h' description='Vehicle Speed Current value': IO_EBS_InputSignals.aVehSpd_Cval_SBSP_0 [-]"; p63 "BlockTend_Stat export=true name=BlockTend_Stat prio=1 dataSetName=std dataClassType=initIO dataClassName=initIO unit='-' description='BlockTend_Stat': IO_EBS_InputSignals.BlockTend_Stat_0 [-]"; p64 "Brake Pedal Position 3 Current value (an CPC3) export=true name=BrkPdlPosn3_Cval prio=1 dataSetName=std dataClassType=initIO dataClassName=initIO unit='%' description='Brake Pedal Position 3 Current value (an CPC3)': IO_EBS_InputSignals.BrkPdlPosn3_Cval_0 [-]"; p65 "Brake Pedal Position 3 Current value (an CPC3) export=true name=BrkPdlPosn3_Cval_SBSP prio=1 dataSetName=std dataClassType=initIO dataClassName=initIO unit='%' description='Brake Pedal Position 3 Current value (an CPC3) SBSP': IO_EBS_InputSignals.BrkPdlPosn3_Cval_SBSP_0 [-]"; p66 "Brake Pedal Position Current value (an CGW) export=true name=BrkPdlPosn_Cval prio=1 dataSetName=std dataClassType=initIO dataClassName=initIO unit='%' description='Brake Pedal Position Current value (an CGW)': IO_EBS_InputSignals.BrkPdlPosn_Cval_0 [-]"; p67 "BrkPress_Rq export=true name=BrkPress_Rq prio=1 dataSetName=std dataClassType=initIO dataClassName=initIO unit='-' description='BrkPress_Rq': IO_EBS_InputSignals.BrkPress_Rq_0 [-]"; p68 "Brake Current value, 254 ERR; 255 SNA; export=true name=BS_Brk_Cval prio=1 dataSetName=std dataClassType=initIO dataClassName=initIO unit='%' description='Brake Current value, 254 ERR; 255 SNA;': IO_EBS_InputSignals.BS_Brk_Cval_0 [-]"; p69 "Brake Current value, 254 ERR; 255 SNA; export=true name=BS_Brk_Cval_SBSP prio=1 dataSetName=std dataClassType=initIO dataClassName=initIO unit='%' description='Brake Current value, 254 ERR; 255 SNA; SBSP': IO_EBS_InputSignals.BS_Brk_Cval_SBSP_0 [-]"; p70 "BS_CS_Acc_Stat export=true name=BS_CS_Acc_Stat prio=1 dataSetName=std dataClassType=initIO dataClassName=initIO unit='-' description='BS_CSCPC_Acc_Stat': IO_EBS_InputSignals.BS_CS_Acc_Stat_0 [-]"; p71 "BS_CS_Acc_Stat_SBSP export=true name=BS_CS_Acc_Stat_SBSP prio=1 dataSetName=std dataClassType=initIO dataClassName=initIO unit='-' description='BS_CSCPC_Acc_Stat': IO_EBS_InputSignals.BS_CS_Acc_Stat_SBSP_0 [-]"; p72 "BS_CS_RqPerf2_Stat export=true name=BS_CS_RqPerf2_Stat prio=1 dataSetName=std dataClassType=initIO dataClassName=initIO unit='-' description='BS_CS_RqPerf2_Stat': IO_EBS_InputSignals.BS_CS_RqPerf2_Stat_0 [-]"; p73 "BS_CS_RqPerf2_Stat_SBSP export=true name=BS_CS_RqPerf2_Stat_SBSP prio=1 dataSetName=std dataClassType=initIO dataClassName=initIO unit='-' description='BS_CS_RqPerf2_Stat_SBSP': IO_EBS_InputSignals.BS_CS_RqPerf2_Stat_SBSP_0 [-]"; p74 "BS_CS_RqPerf_Stat_SBSP export=true name=BS_CS_RqPerf_Stat_SBSP prio=1 dataSetName=std dataClassType=initIO dataClassName=initIO unit='-' description='BS_CS_RqPerf_Stat_SBSP': IO_EBS_InputSignals.BS_CS_RqPerf_Stat_SBSP_0 [-]"; p75 "BS_CSCPC_Acc_Stat export=true name=BS_CSCPC_Acc_Stat prio=1 dataSetName=std dataClassType=initIO dataClassName=initIO unit='-' description='BS_CSCPC_Acc_Stat': IO_EBS_InputSignals.BS_CSCPC_Acc_Stat_0 [-]"; p76 "BS_CSCPC_Acc_Stat_SBSP export=true name=BS_CSCPC_Acc_Stat_SBSP prio=1 dataSetName=std dataClassType=initIO dataClassName=initIO unit='-' description='BS_CSCPC_Acc_Stat_SBSP': IO_EBS_InputSignals.BS_CSCPC_Acc_Stat_SBSP_0 [-]"; p77 "BS_CSCPC_Intf_Stat export=true name=BS_CSCPC_Intf_Stat prio=1 dataSetName=std dataClassType=initIO dataClassName=initIO unit='-' description='BS_CSCPC_Intf_Stat': IO_EBS_InputSignals.BS_CSCPC_Intf_Stat_0 [-]"; p78 "BS_CSCPC_RqPerf_Stat export=true name=BS_CSCPC_RqPerf_Stat prio=1 dataSetName=std dataClassType=initIO dataClassName=initIO unit='-' description='BS_CSCPC_RqPerf_Stat': IO_EBS_InputSignals.BS_CSCPC_RqPerf_Stat_0 [-]"; p79 "BS_HB_Acc_Stat_SBSP export=true name=BS_HB_Acc_Stat_SBSP prio=1 dataSetName=std dataClassType=initIO dataClassName=initIO unit='-' description='BS_HB_Acc_Stat_SBSP': IO_EBS_InputSignals.BS_HB_Acc_Stat_SBSP_0 [-]"; p80 "Brake Current value, 254 ERR; 255 SNA; export=true name=BS_HB_RqPerf_Stat prio=1 dataSetName=std dataClassType=initIO dataClassName=initIO unit='-' description='Brake Current value, 254 ERR; 255 SNA;': IO_EBS_InputSignals.BS_HB_RqPerf_Stat_0 [-]"; p81 "Brake Current value, 254 ERR; 255 SNA; export=true name=BS_HB_RqPerf_Stat_SBSP prio=1 dataSetName=std dataClassType=initIO dataClassName=initIO unit='-' description='Brake Current value, 254 ERR; 255 SNA; SBSP': IO_EBS_InputSignals.BS_HB_RqPerf_Stat_SBSP_0 [-]"; p82 "BS_HBCPC_Acc_Stat_SBSP export=true name=BS_HBCPC_Acc_Stat_SBSP prio=1 dataSetName=std dataClassType=initIO dataClassName=initIO unit='-' description='BS_HBCPC_Acc_Stat_SBSP': IO_EBS_InputSignals.BS_HBCPC_Acc_Stat_SBSP_0 [-]"; p83 "BS_HBCPC_RqPerf_Stat_SBSP export=true name=BS_HBCPC_RqPerf_Stat_SBSP prio=1 dataSetName=std dataClassType=initIO dataClassName=initIO unit='-' description='BS_HBCPC_RqPerf_Stat_SBSP': IO_EBS_InputSignals.BS_HBCPC_RqPerf_Stat_SBSP_0 [-]"; p84 "Road inclination current value (calculated), 254 ERR; 255 SNA; export=true name=BS_RoadIncln_Cval prio=1 dataSetName=std dataClassType=initIO dataClassName=initIO unit='%' description='Road inclination current value (calculated), 254 ERR; 255 SNA;': IO_EBS_InputSignals.BS_RoadIncln_Cval_0 [-]"; p85 "BS_SS_Acc_Stat export=true name=BS_SS_Acc_Stat prio=1 dataSetName=std dataClassType=initIO dataClassName=initIO unit='-' description='BS_CSCPC_Acc_Stat': IO_EBS_InputSignals.BS_SS_Acc_Stat_0 [-]"; p86 "BS_SS_Acc_Stat_SBSP export=true name=BS_SS_Acc_Stat_SBSP prio=1 dataSetName=std dataClassType=initIO dataClassName=initIO unit='-' description='BS_CSCPC_Acc_Stat': IO_EBS_InputSignals.BS_SS_Acc_Stat_SBSP_0 [-]"; p87 "BS_SS_RqPerf_Stat export=true name=BS_SS_RqPerf_Stat prio=1 dataSetName=std dataClassType=initIO dataClassName=initIO unit='-' description='BS_SS_RqPerf_Stat': IO_EBS_InputSignals.BS_SS_RqPerf_Stat_0 [-]"; p88 "BS_SS_RqPerf_Stat_SBSP export=true name=BS_SS_RqPerf_Stat_SBSP prio=1 dataSetName=std dataClassType=initIO dataClassName=initIO unit='-' description='BS_SS_RqPerf_Stat_SBSP': IO_EBS_InputSignals.BS_SS_RqPerf_Stat_SBSP_0 [-]"; p89 "Clutch_Stat_CPC (init) export=true name=Clutch_Stat_CPC prio=1 dataSetName=std dataClassType=initIO dataClassName=initIO unit='-' description='Clutch_Stat_CPC (init)': IO_EBS_InputSignals.Clutch_Stat_CPC_0 [-]"; p90 "ConfLatAccel_SBSP (init) export=true name=ConfLatAccel_SBSP prio=1 dataSetName=std dataClassType=initIO dataClassName=initIO unit='%' description='ConfLatAccel_SBSP': IO_EBS_InputSignals.ConfLatAccel_SBSP_0 [-]"; p91 "ConfLgtAccel_SBSP (init) export=true name=ConfLgtAccel_SBSP prio=1 dataSetName=std dataClassType=initIO dataClassName=initIO unit='%' description='ConfLgtAccel_SBSP': IO_EBS_InputSignals.ConfLgtAccel_SBSP_0 [-]"; p92 "ConfYawRate_SBSP (init) export=true name=ConfYawRate_SBSP prio=1 dataSetName=std dataClassType=initIO dataClassName=initIO unit='%' description='ConfYawRate_SBSP': IO_EBS_InputSignals.ConfYawRate_SBSP_0 [-]"; p93 "drv_BrkPdl_pos export=true name=drv_BrkPdl_pos prio=1 dataSetName=std dataClassType=initIO dataClassName=initIO unit='-' description='drv_BrkPdl_pos': IO_EBS_InputSignals.drv_BrkPdl_pos_0 [-]"; p94 "drv_PkBrk export=true name=drv_PkBrk prio=1 dataSetName=std dataClassType=initIO dataClassName=initIO unit='-' description='drv_PkBrk': IO_EBS_InputSignals.drv_PkBrk_0 [-]"; p95 "ebs_ActlEmotTrq_Nm export=true name=ebs_ActlEmotTrq_Nm prio=1 dataSetName=std dataClassType=initIO dataClassName=initIO unit=Nm description='ebs_ActlEmotTrq_Nm': IO_EBS_InputSignals.ebs_ActlEmotTrq_Nm_0 [-]"; p96 "ebs_ActlEngTrq_Nm export=true name=ebs_ActlEngTrq_Nm prio=1 dataSetName=std dataClassType=initIO dataClassName=initIO unit=Nm description='ebs_ActlEngTrq_Nm': IO_EBS_InputSignals.ebs_ActlEngTrq_Nm_0 [-]"; p97 "ebs_ActlRetTrq_Nm export=true name=ebs_ActlRetTrq_Nm prio=1 dataSetName=std dataClassType=initIO dataClassName=initIO unit=Nm description='ebs_ActlRetTrq_Nm': IO_EBS_InputSignals.ebs_ActlRetTrq_Nm_0 [-]"; p98 "ebs_AdditionalAxle_left_pDmd (init) export=true name=ebs_AdditionalAxle_left_pDmd prio=1 dataSetName=std dataClassType=initIO dataClassName=initIO unit='-' description='ebs_AdditionalAxle_left_pDmd': IO_EBS_InputSignals.ebs_AdditionalAxle_left_pDmd_0 [-]"; p99 "ebs_AdditionalAxle_right_pDmd (init) export=true name=ebs_AdditionalAxle_right_pDmd prio=1 dataSetName=std dataClassType=initIO dataClassName=initIO unit='-' description='ebs_AdditionalAxle_right_pDmd': IO_EBS_InputSignals.ebs_AdditionalAxle_right_pDmd_0 [-]"; p100 "EBS Brake Switch 2 Request state for DTR+, 0 NPSD; 1 PSD; 2 ERR; 3 SNA; export=true name=EBS_BrkSw2_Rq prio=1 dataSetName=std dataClassType=initIO dataClassName=initIO unit='-' description='EBS Brake Switch 2 Request state for DTR+, 0 NPSD; 1 PSD; 2 ERR; 3 SNA;': IO_EBS_InputSignals.EBS_BrkSw2_Rq_0 [-]"; p101 "EBS Brake Switch 2 Request state for DTR+, 0 NPSD; 1 PSD; 2 ERR; 3 SNA; export=true name=EBS_BrkSw2_Rq_SBSP prio=1 dataSetName=std dataClassType=initIO dataClassName=initIO unit='-' description='EBS Brake Switch 2 Request state for DTR+, 0 NPSD; 1 PSD; 2 ERR; 3 SNA;': IO_EBS_InputSignals.EBS_BrkSw2_Rq_SBSP_0 [-]"; p102 "ebs_ESCsens_y_acceleration export=true name=ebs_ESCsens_y_acceleration prio=1 dataSetName=std dataClassType=initIO dataClassName=initIO unit='m/s^2' description='ebs_ESCsens_y_acceleration': IO_EBS_InputSignals.ebs_ESCsens_y_acceleration_0 [-]"; p103 "ebs_FrontAxle_left_pDmd (init) export=true name=ebs_FrontAxle_left_pDmd prio=1 dataSetName=std dataClassType=initIO dataClassName=initIO unit='-' description='ebs_FrontAxle_left_pDmd': IO_EBS_InputSignals.ebs_FrontAxle_left_pDmd_0 [-]"; p104 "ebs_FrontAxle_right_pDmd (init) export=true name=ebs_FrontAxle_right_pDmd prio=1 dataSetName=std dataClassType=initIO dataClassName=initIO unit='-' description='ebs_FrontAxle_right_pDmd': IO_EBS_InputSignals.ebs_FrontAxle_right_pDmd_0 [-]"; p105 "ebs_i_Emot export=true name=ebs_i_Emot prio=1 dataSetName=std dataClassType=initIO dataClassName=initIO unit='-' description='ebs_i_Emot': IO_EBS_InputSignals.ebs_i_Emot_0 [-]"; p106 "ebs_i_Ret export=true name=ebs_i_Ret prio=1 dataSetName=std dataClassType=initIO dataClassName=initIO unit='-' description='ebs_i_Ret': IO_EBS_InputSignals.ebs_i_Ret_0 [-]"; p107 "ebs_kappa export=true name=ebs_kappa prio=1 dataSetName=std dataClassType=initIO dataClassName=initIO unit='-' description='ebs_kappa': IO_EBS_InputSignals.ebs_kappa_0 [-]"; p108 "ebs_RearAxle_left_pDmd (init) export=true name=ebs_RearAxle_left_pDmd prio=1 dataSetName=std dataClassType=initIO dataClassName=initIO unit='-' description='ebs_RearAxle_left_pDmd': IO_EBS_InputSignals.ebs_RearAxle_left_pDmd_0 [-]"; p109 "ebs_RearAxle_right_pDmd (init) export=true name=ebs_RearAxle_right_pDmd prio=1 dataSetName=std dataClassType=initIO dataClassName=initIO unit='-' description='ebs_RearAxle_right_pDmd': IO_EBS_InputSignals.ebs_RearAxle_right_pDmd_0 [-]"; p110 "ebs_sBSP_stABSInValve_Addl_Left export=true name=ebs_sBSP_stABSInValve_Addl_Left prio=1 dataSetName=std dataClassType=initIO dataClassName=initIO unit='-' description='ebs_sBSP_stABSInValve_Addl_Left': IO_EBS_InputSignals.ebs_sBSP_stABSInValve_Addl_Left_0 [-]"; p111 "ebs_sBSP_stABSInValve_Addl_Right export=true name=ebs_sBSP_stABSInValve_Addl_Right prio=1 dataSetName=std dataClassType=initIO dataClassName=initIO unit='-' description='ebs_sBSP_stABSInValve_Addl_Right': IO_EBS_InputSignals.ebs_sBSP_stABSInValve_Addl_Right_0 [-]"; p112 "ebs_sBSP_stABSInValve_Front_Left export=true name=ebs_sBSP_stABSInValve_Front_Left prio=1 dataSetName=std dataClassType=initIO dataClassName=initIO unit='-' description='ebs_sBSP_stABSInValve_Front_Left': IO_EBS_InputSignals.ebs_sBSP_stABSInValve_Front_Left_0 [-]"; p113 "ebs_sBSP_stABSInValve_Front_Right export=true name=ebs_sBSP_stABSInValve_Front_Right prio=1 dataSetName=std dataClassType=initIO dataClassName=initIO unit='-' description='ebs_sBSP_stABSInValve_Front_Right': IO_EBS_InputSignals.ebs_sBSP_stABSInValve_Front_Right_0 [-]"; p114 "ebs_sBSP_stABSInValve_RCMax_Front (init),   export=true name=ebs_sBSP_stABSInValve_RCMax_Front prio=1 dataSetName=std dataClassType=initIO dataClassName=initIO unit='-' description=' ': IO_EBS_InputSignals.ebs_sBSP_stABSInValve_RCMax_Front_0 [-]"; p115 "ebs_sBSP_stABSInValve_RCMax_Rear (init),   export=true name=ebs_sBSP_stABSInValve_RCMax_Rear prio=1 dataSetName=std dataClassType=initIO dataClassName=initIO unit='-' description=' ': IO_EBS_InputSignals.ebs_sBSP_stABSInValve_RCMax_Rear_0 [-]"; p116 "ebs_sBSP_stABSInValve_Rear_Left export=true name=ebs_sBSP_stABSInValve_Rear_Left prio=1 dataSetName=std dataClassType=initIO dataClassName=initIO unit='-' description='ebs_sBSP_stABSInValve_Rear_Left': IO_EBS_InputSignals.ebs_sBSP_stABSInValve_Rear_Left_0 [-]"; p117 "ebs_sBSP_stABSInValve_Rear_Right export=true name=ebs_sBSP_stABSInValve_Rear_Right prio=1 dataSetName=std dataClassType=initIO dataClassName=initIO unit='-' description='ebs_sBSP_stABSInValve_Rear_Right': IO_EBS_InputSignals.ebs_sBSP_stABSInValve_Rear_Right_0 [-]"; p118 "ebs_sBSP_stABSOutValve_Addl_Left export=true name=ebs_sBSP_stABSOutValve_Addl_Left prio=1 dataSetName=std dataClassType=initIO dataClassName=initIO unit='-' description='ebs_sBSP_stABSOutValve_Addl_Left': IO_EBS_InputSignals.ebs_sBSP_stABSOutValve_Addl_Left_0 [-]"; p119 "ebs_sBSP_stABSOutValve_Addl_Right export=true name=ebs_sBSP_stABSOutValve_Addl_Right prio=1 dataSetName=std dataClassType=initIO dataClassName=initIO unit='-' description='ebs_sBSP_stABSOutValve_Addl_Right': IO_EBS_InputSignals.ebs_sBSP_stABSOutValve_Addl_Right_0 [-]"; p120 "ebs_sBSP_stABSOutValve_Front_Left export=true name=ebs_sBSP_stABSOutValve_Front_Left prio=1 dataSetName=std dataClassType=initIO dataClassName=initIO unit='-' description='ebs_sBSP_stABSOutValve_Front_Left': IO_EBS_InputSignals.ebs_sBSP_stABSOutValve_Front_Left_0 [-]"; p121 "ebs_sBSP_stABSOutValve_Front_Right export=true name=ebs_sBSP_stABSOutValve_Front_Right prio=1 dataSetName=std dataClassType=initIO dataClassName=initIO unit='-' description='ebs_sBSP_stABSOutValve_Front_Right': IO_EBS_InputSignals.ebs_sBSP_stABSOutValve_Front_Right_0 [-]"; p122 "ebs_sBSP_stABSOutValve_RCMax_Front (init),   export=true name=ebs_sBSP_stABSOutValve_RCMax_Front prio=1 dataSetName=std dataClassType=initIO dataClassName=initIO unit='-' description=' ': IO_EBS_InputSignals.ebs_sBSP_stABSOutValve_RCMax_Front_0 [-]"; p123 "ebs_sBSP_stABSOutValve_RCMax_Rear (init),   export=true name=ebs_sBSP_stABSOutValve_RCMax_Rear prio=1 dataSetName=std dataClassType=initIO dataClassName=initIO unit='-' description=' ': IO_EBS_InputSignals.ebs_sBSP_stABSOutValve_RCMax_Rear_0 [-]"; p124 "ebs_sBSP_stABSOutValve_Rear_Left export=true name=ebs_sBSP_stABSOutValve_Rear_Left prio=1 dataSetName=std dataClassType=initIO dataClassName=initIO unit='-' description='ebs_sBSP_stABSOutValve_Rear_Left': IO_EBS_InputSignals.ebs_sBSP_stABSOutValve_Rear_Left_0 [-]"; p125 "ebs_sBSP_stABSOutValve_Rear_Right export=true name=ebs_sBSP_stABSOutValve_Rear_Right prio=1 dataSetName=std dataClassType=initIO dataClassName=initIO unit='-' description='ebs_sBSP_stABSOutValve_Rear_Right': IO_EBS_InputSignals.ebs_sBSP_stABSOutValve_Rear_Right_0 [-]"; p126 "ebs_sBSP_stAPCVBuValve export=true name=ebs_sBSP_stAPCVBuValve prio=1 dataSetName=std dataClassType=initIO dataClassName=initIO unit='-' description='ebs_sBSP_stAPCVBuValve': IO_EBS_InputSignals.ebs_sBSP_stAPCVBuValve_0 [-]"; p127 "ebs_sBSP_stAxmoBuValve export=true name=ebs_sBSP_stAxmoBuValve prio=1 dataSetName=std dataClassType=initIO dataClassName=initIO unit='-' description='ebs_sBSP_stAxmoBuValve': IO_EBS_InputSignals.ebs_sBSP_stAxmoBuValve_0 [-]"; p128 "ebs_sBSP_stCMaxBuValve export=true name=ebs_sBSP_stCMaxBuValve prio=1 dataSetName=std dataClassType=initIO dataClassName=initIO unit='-' description='ebs_sBSP_stCMaxBuValve': IO_EBS_InputSignals.ebs_sBSP_stCMaxBuValve_0 [-]"; p129 "ebs_SumBrakingForces_Trailer (init) export=true name=ebs_SumBrakingForces_Trailer prio=1 dataSetName=std dataClassType=initIO dataClassName=initIO unit='-' description='ebs_SumBrakingForces_Trailer': IO_EBS_InputSignals.ebs_SumBrakingForces_Trailer_0 [-]"; p130 "ebs_SumBrakingForces_Vehicle (init) export=true name=ebs_SumBrakingForces_Vehicle prio=1 dataSetName=std dataClassType=initIO dataClassName=initIO unit='-' description='ebs_SumBrakingForces_Vehicle': IO_EBS_InputSignals.ebs_SumBrakingForces_Vehicle_0 [-]"; p131 "ebs_TCV_pDmd (init) export=true name=ebs_TCV_pDmd prio=1 dataSetName=std dataClassType=initIO dataClassName=initIO unit='-' description='ebs_TCV_pDmd': IO_EBS_InputSignals.ebs_TCV_pDmd_0 [-]"; p132 "ebs_zReqBrake export=true name=ebs_zReqBrake prio=1 dataSetName=std dataClassType=initIO dataClassName=initIO unit='-' description='ebs_zReqBrake': IO_EBS_InputSignals.ebs_zReqBrake_0 [-]"; p133 "ebs_zReqEB export=true name=ebs_zReqEB prio=1 dataSetName=std dataClassType=initIO dataClassName=initIO unit='-' description='ebs_zReqEB': IO_EBS_InputSignals.ebs_zReqEB_0 [-]"; p134 "ebs_zRet export=true name=ebs_zRet prio=1 dataSetName=std dataClassType=initIO dataClassName=initIO unit='-' description='ebs_zRet': IO_EBS_InputSignals.ebs_zRet_0 [-]"; p135 "ebs_zSlopeComp export=true name=ebs_zSlopeComp prio=1 dataSetName=std dataClassType=initIO dataClassName=initIO unit='-' description='ebs_zSlopeComp': IO_EBS_InputSignals.ebs_zSlopeComp_0 [-]"; p136 "ebs_zSoll_BWG export=true name=ebs_zSoll_BWG prio=1 dataSetName=std dataClassType=initIO dataClassName=initIO unit='-' description='ebs_zSoll_BWG': IO_EBS_InputSignals.ebs_zSoll_BWG_0 [-]"; p137 "EdrvRefTrq_Cval (init) export=true name=EdrvRefTrq_Cval prio=1 dataSetName=std dataClassType=initIO dataClassName=initIO unit='-' description='EdrvRefTrq_Cval (init)': IO_EBS_InputSignals.EdrvRefTrq_Cval_0 [-]"; p138 "EngPctTrqActl_Cval export=true name=EngPctTrqActl_Cval prio=1 dataSetName=std dataClassType=initIO dataClassName=initIO unit='-' description='EngPctTrqActl_Cval': IO_EBS_InputSignals.EngPctTrqActl_Cval_0 [-]"; p139 "EngRefTrq_Cval export=true name=EngRefTrq_Cval prio=1 dataSetName=std dataClassType=initIO dataClassName=initIO unit='-' description='EngRefTrq_Cval': IO_EBS_InputSignals.EngRefTrq_Cval_0 [-]"; p140 "EngRetTrqMax_Rq (toCAN) export=true name=EngRetTrqMax_Rq prio=1 dataSetName=std dataClassType=initIO dataClassName=initIO unit='-' description='EngRetTrqMax_Rq (toCAN)': IO_EBS_InputSignals.EngRetTrqMax_Rq_0 [-]"; p141 "EngRetTrqMin_Rq (to CAN) export=true name=EngRetTrqMin_Rq prio=1 dataSetName=std dataClassType=initIO dataClassName=initIO unit='-' description='EngRetTrqMin_Rq (to CAN)': IO_EBS_InputSignals.EngRetTrqMin_Rq_0 [-]"; p142 "Engine RPM Current value from CPC export=true name=EngRPM_Cval_CPC3 prio=1 dataSetName=std dataClassType=initIO dataClassName=initIO unit='-' description='Engine RPM Current value from CPC': IO_EBS_InputSignals.EngRPM_Cval_CPC3_0 [-]"; p143 "curvature of road [1/m] export=true name=env_curv_pm prio=1 dataSetName=std dataClassType=initIO dataClassName=initIO unit='-' description='curvature of road [1/m]': IO_EBS_InputSignals.env_curv_pm_0 [-]"; p144 "slope of road [%] export=true name=env_road_slope_pct prio=1 dataSetName=std dataClassType=initIO dataClassName=initIO unit='-' description='slope of road [%]': IO_EBS_InputSignals.env_road_slope_pct_0 [-]"; p145 "ExtAccel_Rq_CPC5ce [m/s^2] export=true name=ExtAccel_Rq_CPC5ce prio=1 dataSetName=std dataClassType=initIO dataClassName=initIO unit='-' description='ExtAccel_Rq_CPC5ce [m/s^2]': IO_EBS_InputSignals.ExtAccel_Rq_CPC5ce_0 [-]"; p146 "ExtAccel_Rq_CPC [m/s^2] export=true name=ExtAccel_Rq_CPC prio=1 dataSetName=std dataClassType=initIO dataClassName=initIO unit='-' description='ExtAccel_Rq_CPC [m/s^2]': IO_EBS_InputSignals.ExtAccel_Rq_CPC_0 [-]"; p147 "ExtAccel_Rq_VRDU3 export=true name=ExtAccel_Rq_VRDU3 prio=1 dataSetName=std dataClassType=initIO dataClassName=initIO unit='m/s^2' description='ACC External Acceleration Demand': IO_EBS_InputSignals.ExtAccel_Rq_VRDU3_0 [-]"; p148 "ExtAccel_Rq_VRDU [m/s^2] export=true name=ExtAccel_Rq_VRDU prio=1 dataSetName=std dataClassType=initIO dataClassName=initIO unit='-' description='ExtAccel_Rq_VRDU [m/s^2]': IO_EBS_InputSignals.ExtAccel_Rq_VRDU_0 [-]"; p149 "ExtBrkStat_Rq_CPC [-] export=true name=ExtBrkStat_Rq_CPC prio=1 dataSetName=std dataClassType=initIO dataClassName=initIO unit='-' description='ExtBrkStat_Rq_CPC [-]': IO_EBS_InputSignals.ExtBrkStat_Rq_CPC_0 [-]"; p150 "ExtBrkStat_Rq_VRDU [-] export=true name=ExtBrkStat_Rq_VRDU prio=1 dataSetName=std dataClassType=initIO dataClassName=initIO unit='-' description='ExtBrkStat_Rq_VRDU [-]': IO_EBS_InputSignals.ExtBrkStat_Rq_VRDU_0 [-]"; p151 "FoundBrk_Stat service brake is:   0 --> inaktive , 1 --> aktive, 4 --> sna export=true name=FoundBrk_Stat prio=1 dataSetName=std dataClassType=initIO dataClassName=initIO unit='-' description='FoundBrk_Stat, service brake is:   0 --> inaktive , 1 --> aktive, 4 --> sna': IO_EBS_InputSignals.FoundBrk_Stat_0 [-]"; p152 "FullBrkAllow_Stat_SBSP export=true name=FullBrkAllow_Stat_SBSP prio=1 dataSetName=std dataClassType=initIO dataClassName=initIO unit='-' description='FullBrkAllow_Stat_SBSP': IO_EBS_InputSignals.FullBrkAllow_Stat_SBSP_0 [-]"; p153 "GroCmbVehWeight_Cval (init) export=true name=GroCmbVehWeight_Cval prio=1 dataSetName=std dataClassType=initIO dataClassName=initIO unit=kg description='GroCmbVehWeight_Cval': IO_EBS_InputSignals.GroCmbVehWeight_Cval_0 [-]"; p154 "HB_Rq_Stat_CPC export=true name=HB_Rq_Stat_CPC prio=1 dataSetName=std dataClassType=initIO dataClassName=initIO unit='-' description='HB_Rq_Stat_CPC': IO_EBS_InputSignals.HB_Rq_Stat_CPC_0 [-]"; p155 "HB_Rq_Stat_VRDU export=true name=HB_Rq_Stat_VRDU prio=1 dataSetName=std dataClassType=initIO dataClassName=initIO unit='-' description='HB_Rq_Stat_VRDU': IO_EBS_InputSignals.HB_Rq_Stat_VRDU_0 [-]"; p156 "Hill Holder Availability Current State, 0 HH_AVL; 1 HH_ACTV_NOT_FF; 2 HH_MF; 3 SNA; export=true name=HillHolderAvl_Stat prio=1 dataSetName=std dataClassType=initIO dataClassName=initIO unit='-' description='Hill Holder Availability Current State, 0 HH_AVL; 1 HH_ACTV_NOT_FF; 2 HH_MF; 3 SNA;': IO_EBS_InputSignals.HillHolderAvl_Stat_0 [-]"; p157 "mec3d_ESCsens_gamma_rate export=true name=mec3d_ESCsens_gamma_rate prio=1 dataSetName=std dataClassType=initIO dataClassName=initIO unit='rad/s' description='mec3d_ESCsens_gamma_rate': IO_EBS_InputSignals.mec3d_ESCsens_gamma_rate_0 [-]"; p158 "mec3d_ESCsens_y_acceleration export=true name=mec3d_ESCsens_y_acceleration prio=1 dataSetName=std dataClassType=initIO dataClassName=initIO unit='m/s^2' description='mec3d_ESCsens_y_acceleration': IO_EBS_InputSignals.mec3d_ESCsens_y_acceleration_0 [-]"; p159 "mec_veh_AxleLoad1 (init) export=true name=mec_veh_AxleLoad1 prio=1 dataSetName=std dataClassType=initIO dataClassName=initIO unit=kg description='mec_veh_AxleLoad1': IO_EBS_InputSignals.mec_veh_AxleLoad1_0 [-]"; p160 "mec_veh_AxleLoad2 (init) export=true name=mec_veh_AxleLoad2 prio=1 dataSetName=std dataClassType=initIO dataClassName=initIO unit=kg description='mec_veh_AxleLoad2': IO_EBS_InputSignals.mec_veh_AxleLoad2_0 [-]"; p161 "mec_veh_AxleLoad3 (init) export=true name=mec_veh_AxleLoad3 prio=1 dataSetName=std dataClassType=initIO dataClassName=initIO unit=kg description='mec_veh_AxleLoad3': IO_EBS_InputSignals.mec_veh_AxleLoad3_0 [-]"; p162 "mec_veh_AxleLoad4 (init) export=true name=mec_veh_AxleLoad4 prio=1 dataSetName=std dataClassType=initIO dataClassName=initIO unit=kg description='mec_veh_AxleLoad4': IO_EBS_InputSignals.mec_veh_AxleLoad4_0 [-]"; p163 "mec_veh_Trailer02AxleLoad1 (init) export=true name=mec_veh_Trailer02AxleLoad1 prio=1 dataSetName=std dataClassType=initIO dataClassName=initIO unit=kg description='mec_veh_Trailer02AxleLoad1': IO_EBS_InputSignals.mec_veh_Trailer02AxleLoad1_0 [-]"; p164 "mec_veh_Trailer02AxleLoad2 (init) export=true name=mec_veh_Trailer02AxleLoad2 prio=1 dataSetName=std dataClassType=initIO dataClassName=initIO unit=kg description='mec_veh_Trailer02AxleLoad2': IO_EBS_InputSignals.mec_veh_Trailer02AxleLoad2_0 [-]"; p165 "mec_veh_Trailer02AxleLoad3 (init) export=true name=mec_veh_Trailer02AxleLoad3 prio=1 dataSetName=std dataClassType=initIO dataClassName=initIO unit=kg description='mec_veh_Trailer02AxleLoad3': IO_EBS_InputSignals.mec_veh_Trailer02AxleLoad3_0 [-]"; p166 "mec_veh_Trailer02AxleLoad4 (init) export=true name=mec_veh_Trailer02AxleLoad4 prio=1 dataSetName=std dataClassType=initIO dataClassName=initIO unit=kg description='mec_veh_Trailer02AxleLoad4': IO_EBS_InputSignals.mec_veh_Trailer02AxleLoad4_0 [-]"; p167 "mec_veh_Trailer02AxleLoad5 (init) export=true name=mec_veh_Trailer02AxleLoad5 prio=1 dataSetName=std dataClassType=initIO dataClassName=initIO unit=kg description='mec_veh_Trailer02AxleLoad5': IO_EBS_InputSignals.mec_veh_Trailer02AxleLoad5_0 [-]"; p168 "mec_veh_Trailer02AxleLoad6 (init) export=true name=mec_veh_Trailer02AxleLoad6 prio=1 dataSetName=std dataClassType=initIO dataClassName=initIO unit=kg description='mec_veh_Trailer02AxleLoad6': IO_EBS_InputSignals.mec_veh_Trailer02AxleLoad6_0 [-]"; p169 "mec_veh_TrailerAxleLoad1 (init) export=true name=mec_veh_TrailerAxleLoad1 prio=1 dataSetName=std dataClassType=initIO dataClassName=initIO unit=kg description='mec_veh_TrailerAxleLoad1': IO_EBS_InputSignals.mec_veh_TrailerAxleLoad1_0 [-]"; p170 "mec_veh_TrailerAxleLoad2 (init) export=true name=mec_veh_TrailerAxleLoad2 prio=1 dataSetName=std dataClassType=initIO dataClassName=initIO unit=kg description='mec_veh_TrailerAxleLoad2': IO_EBS_InputSignals.mec_veh_TrailerAxleLoad2_0 [-]"; p171 "mec_veh_TrailerAxleLoad3 (init) export=true name=mec_veh_TrailerAxleLoad3 prio=1 dataSetName=std dataClassType=initIO dataClassName=initIO unit=kg description='mec_veh_TrailerAxleLoad3': IO_EBS_InputSignals.mec_veh_TrailerAxleLoad3_0 [-]"; p172 "mec_veh_transVel export=true name=mec_veh_transVel prio=1 dataSetName=std dataClassType=initIO dataClassName=initIO unit='-' description='mec_veh_transVel': IO_EBS_InputSignals.mec_veh_transVel_0 [-]"; p173 "MinAvlEmotTrq_Cval_CPC (init) export=true name=MinAvlEmotTrq_Cval_CPC prio=1 dataSetName=std dataClassType=initIO dataClassName=initIO unit='-' description='MinAvlEmotTrq_Cval_CPC (init)': IO_EBS_InputSignals.MinAvlEmotTrq_Cval_CPC_0 [-]"; p174 "NomFrictEngPctTrq_Cval export=true name=NomFrictEngPctTrq_Cval prio=1 dataSetName=std dataClassType=initIO dataClassName=initIO unit='-' description='NomFrictEngPctTrq_Cval': IO_EBS_InputSignals.NomFrictEngPctTrq_Cval_0 [-]"; p175 "NrTrlr_Stat_SBSP (init) export=true name=NrTrlr_Stat_SBSP prio=1 dataSetName=std dataClassType=initIO dataClassName=initIO unit='' description='NrTrlr_Stat_SBSP': IO_EBS_InputSignals.NrTrlr_Stat_SBSP_0 [-]"; p176 "PkBrk_Rq_VRDU export=true name=PkBrk_Rq_VRDU prio=1 dataSetName=std dataClassType=initIO dataClassName=initIO unit='-' description='PkBrk_Rq_VRDU': IO_EBS_InputSignals.PkBrk_Rq_VRDU_0 [-]"; p177 "Front axle: acting pressure export=true name=pne_brk_AdditionalAxle_left_pAct prio=1 dataSetName=std dataClassType=initIO dataClassName=initIO unit='bar' description='actual pressure Additional leftt at 2k-AXMO': IO_EBS_InputSignals.pne_brk_AdditionalAxle_left_pAct_0 [-]"; p178 "Front axle: acting pressure export=true name=pne_brk_AdditionalAxle_right_pAct prio=1 dataSetName=std dataClassType=initIO dataClassName=initIO unit='bar' description='actual pressure Additional right at 2k-AXMO': IO_EBS_InputSignals.pne_brk_AdditionalAxle_right_pAct_0 [-]"; p179 "pne_brk_Axle1_BrakingForce_at8p5bar [N] (init) export=true name=pne_brk_Axle1_BrakingForce_at8p5bar prio=1 dataSetName=std dataClassType=initIO dataClassName=initIO unit=N description='pne_brk_Axle1_BrakingForce_at8p5bar [N] (init)': IO_EBS_InputSignals.pne_brk_Axle1_BrakingForce_at8p5bar_0 [-]"; p180 "axle 1 left temperature of the friction area [degC] (init) export=true name=pne_brk_Axle1_left_Tinterior prio=1 dataSetName=std dataClassType=initIO dataClassName=initIO unit=degC description='axle 1 left inner temperature [degC] (init)': IO_EBS_InputSignals.pne_brk_Axle1_left_Tinterior_0 [-]"; p181 "axle 1 right temperature of the friction area [degC] (init) export=true name=pne_brk_Axle1_right_Tinterior prio=1 dataSetName=std dataClassType=initIO dataClassName=initIO unit=degC description='axle 1 right inner temperature [degC] (init)': IO_EBS_InputSignals.pne_brk_Axle1_right_Tinterior_0 [-]"; p182 "pne_brk_Axle1_torque_sns export=true name=pne_brk_Axle1_torque_sns prio=1 dataSetName=std dataClassType=initIO dataClassName=initIO unit='-' description='pne_brk_Axle1_torque_sns': IO_EBS_InputSignals.pne_brk_Axle1_torque_sns_0 [-]"; p183 "pne_brk_Axle2_BrakingForce_at8p5bar [N] (init) export=true name=pne_brk_Axle2_BrakingForce_at8p5bar prio=1 dataSetName=std dataClassType=initIO dataClassName=initIO unit=N description='pne_brk_Axle2_BrakingForce_at8p5bar [N] (init)': IO_EBS_InputSignals.pne_brk_Axle2_BrakingForce_at8p5bar_0 [-]"; p184 "axle 2 left temperature of the friction area [degC] (init) export=true name=pne_brk_Axle2_left_Tinterior prio=1 dataSetName=std dataClassType=initIO dataClassName=initIO unit=degC description='axle 1 left inner temperature [degC] (init)': IO_EBS_InputSignals.pne_brk_Axle2_left_Tinterior_0 [-]"; p185 "axle 2 right temperature of the friction area [degC] (init) export=true name=pne_brk_Axle2_right_Tinterior prio=1 dataSetName=std dataClassType=initIO dataClassName=initIO unit=degC description='axle 1 right inner temperature [degC] (init)': IO_EBS_InputSignals.pne_brk_Axle2_right_Tinterior_0 [-]"; p186 "pne_brk_Axle2_torque_sns export=true name=pne_brk_Axle2_torque_sns prio=1 dataSetName=std dataClassType=initIO dataClassName=initIO unit='-' description='pne_brk_Axle2_torque_sns': IO_EBS_InputSignals.pne_brk_Axle2_torque_sns_0 [-]"; p187 "pne_brk_Axle3_BrakingForce_at8p5bar [N] (init) export=true name=pne_brk_Axle3_BrakingForce_at8p5bar prio=1 dataSetName=std dataClassType=initIO dataClassName=initIO unit=N description='pne_brk_Axle3_BrakingForce_at8p5bar [N] (init)': IO_EBS_InputSignals.pne_brk_Axle3_BrakingForce_at8p5bar_0 [-]"; p188 "axle 3 left temperature of the friction area [degC] (init) export=true name=pne_brk_Axle3_left_Tinterior prio=1 dataSetName=std dataClassType=initIO dataClassName=initIO unit=degC description='axle 1 left inner temperature [degC] (init)': IO_EBS_InputSignals.pne_brk_Axle3_left_Tinterior_0 [-]"; p189 "axle 3 right temperature of the friction area [degC] (init) export=true name=pne_brk_Axle3_right_Tinterior prio=1 dataSetName=std dataClassType=initIO dataClassName=initIO unit=degC description='axle 1 right inner temperature [degC] (init)': IO_EBS_InputSignals.pne_brk_Axle3_right_Tinterior_0 [-]"; p190 "pne_brk_Axle3_torque_sns export=true name=pne_brk_Axle3_torque_sns prio=1 dataSetName=std dataClassType=initIO dataClassName=initIO unit='-' description='pne_brk_Axle3_torque_sns': IO_EBS_InputSignals.pne_brk_Axle3_torque_sns_0 [-]"; p191 "pne_brk_Axle4_BrakingForce_at8p5bar [N] (init) export=true name=pne_brk_Axle4_BrakingForce_at8p5bar prio=1 dataSetName=std dataClassType=initIO dataClassName=initIO unit=N description='pne_brk_Axle4_BrakingForce_at8p5bar [N] (init)': IO_EBS_InputSignals.pne_brk_Axle4_BrakingForce_at8p5bar_0 [-]"; p192 "axle 4 left temperature of the friction area [degC] (init) export=true name=pne_brk_Axle4_left_Tinterior prio=1 dataSetName=std dataClassType=initIO dataClassName=initIO unit=degC description='axle 1 left inner temperature [degC] (init)': IO_EBS_InputSignals.pne_brk_Axle4_left_Tinterior_0 [-]"; p193 "axle 4 right temperature of the friction area [degC] (init) export=true name=pne_brk_Axle4_right_Tinterior prio=1 dataSetName=std dataClassType=initIO dataClassName=initIO unit=degC description='axle 1 right inner temperature [degC] (init)': IO_EBS_InputSignals.pne_brk_Axle4_right_Tinterior_0 [-]"; p194 "pne_brk_Axle4_torque_sns export=true name=pne_brk_Axle4_torque_sns prio=1 dataSetName=std dataClassType=initIO dataClassName=initIO unit='-' description='pne_brk_Axle4_torque_sns': IO_EBS_InputSignals.pne_brk_Axle4_torque_sns_0 [-]"; p195 "Front axle: acting pressure export=true name=pne_brk_FrontAxle_pAct prio=1 dataSetName=std dataClassType=initIO dataClassName=initIO unit='bar' description='Front axle: acting pressure': IO_EBS_InputSignals.pne_brk_FrontAxle_pAct_0 [-]"; p196 "Rear axle left: acting pressure export=true name=pne_brk_RearAxle_left_pAct prio=1 dataSetName=std dataClassType=initIO dataClassName=initIO unit='bar' description='Rear axle left: acting pressure': IO_EBS_InputSignals.pne_brk_RearAxle_left_pAct_0 [-]"; p197 "Rear axle right: acting pressure export=true name=pne_brk_RearAxle_right_pAct prio=1 dataSetName=std dataClassType=initIO dataClassName=initIO unit='bar' description='Rear axle right: acting pressure': IO_EBS_InputSignals.pne_brk_RearAxle_right_pAct_0 [-]"; p198 "wheel speed additional left wheel export=true name=pne_brk_rotVel_al prio=1 dataSetName=std dataClassType=initIO dataClassName=initIO unit='-' description='wheel speed additional left wheel': IO_EBS_InputSignals.pne_brk_rotVel_al_0 [-]"; p199 "wheel speed additional right wheel export=true name=pne_brk_rotVel_ar prio=1 dataSetName=std dataClassType=initIO dataClassName=initIO unit='-' description='wheel speed additional right wheel': IO_EBS_InputSignals.pne_brk_rotVel_ar_0 [-]"; p200 "wheel speed front left wheel export=true name=pne_brk_rotVel_fl prio=1 dataSetName=std dataClassType=initIO dataClassName=initIO unit='-' description='wheel speed front left wheel': IO_EBS_InputSignals.pne_brk_rotVel_fl_0 [-]"; p201 "wheel speed front right wheel export=true name=pne_brk_rotVel_fr prio=1 dataSetName=std dataClassType=initIO dataClassName=initIO unit='-' description='wheel speed front right wheel': IO_EBS_InputSignals.pne_brk_rotVel_fr_0 [-]"; p202 "wheel speed rear left wheel export=true name=pne_brk_rotVel_rl prio=1 dataSetName=std dataClassType=initIO dataClassName=initIO unit='-' description='wheel speed rear left wheel': IO_EBS_InputSignals.pne_brk_rotVel_rl_0 [-]"; p203 "wheel speed rear right wheel export=true name=pne_brk_rotVel_rr prio=1 dataSetName=std dataClassType=initIO dataClassName=initIO unit='-' description='wheel speed rear right wheel': IO_EBS_InputSignals.pne_brk_rotVel_rr_0 [-]"; p204 "Front axle: acting pressure export=true name=pne_brk_TCV_pAct prio=1 dataSetName=std dataClassType=initIO dataClassName=initIO unit='bar' description='actual pressure TCV': IO_EBS_InputSignals.pne_brk_TCV_pAct_0 [-]"; p205 "pne_brk_Trailer02Axle1_BrakingForce_at8p5bar [N] (init) export=true name=pne_brk_Trailer02Axle1_BrakingForce_at8p5bar prio=1 dataSetName=std dataClassType=initIO dataClassName=initIO unit=N description='pne_brk_Trailer02Axle1_BrakingForce_at8p5bar [N] (init)': IO_EBS_InputSignals.pne_brk_Trailer02Axle1_BrakingForce_at8p5bar_0 [-]"; p206 "pne_brk_Trailer02Axle1_torque_sns (init) export=true name=pne_brk_Trailer02Axle1_torque_sns prio=1 dataSetName=std dataClassType=initIO dataClassName=initIO unit=kg description='pne_brk_Trailer02Axle1_torque_sns': IO_EBS_InputSignals.pne_brk_Trailer02Axle1_torque_sns_0 [-]"; p207 "pne_brk_Trailer02Axle2_BrakingForce_at8p5bar [N] (init) export=true name=pne_brk_Trailer02Axle2_BrakingForce_at8p5bar prio=1 dataSetName=std dataClassType=initIO dataClassName=initIO unit=N description='pne_brk_Trailer02Axle2_BrakingForce_at8p5bar [N] (init)': IO_EBS_InputSignals.pne_brk_Trailer02Axle2_BrakingForce_at8p5bar_0 [-]"; p208 "pne_brk_Trailer02Axle2_torque_sns (init) export=true name=pne_brk_Trailer02Axle2_torque_sns prio=1 dataSetName=std dataClassType=initIO dataClassName=initIO unit=kg description='pne_brk_Trailer02Axle2_torque_sns': IO_EBS_InputSignals.pne_brk_Trailer02Axle2_torque_sns_0 [-]"; p209 "pne_brk_Trailer02Axle3_BrakingForce_at8p5bar [N] (init) export=true name=pne_brk_Trailer02Axle3_BrakingForce_at8p5bar prio=1 dataSetName=std dataClassType=initIO dataClassName=initIO unit=N description='pne_brk_Trailer02Axle3_BrakingForce_at8p5bar [N] (init)': IO_EBS_InputSignals.pne_brk_Trailer02Axle3_BrakingForce_at8p5bar_0 [-]"; p210 "pne_brk_Trailer02Axle3_torque_sns (init) export=true name=pne_brk_Trailer02Axle3_torque_sns prio=1 dataSetName=std dataClassType=initIO dataClassName=initIO unit=kg description='pne_brk_Trailer02Axle3_torque_sns': IO_EBS_InputSignals.pne_brk_Trailer02Axle3_torque_sns_0 [-]"; p211 "pne_brk_Trailer02Axle4_BrakingForce_at8p5bar [N] (init) export=true name=pne_brk_Trailer02Axle4_BrakingForce_at8p5bar prio=1 dataSetName=std dataClassType=initIO dataClassName=initIO unit=N description='pne_brk_Trailer02Axle4_BrakingForce_at8p5bar [N] (init)': IO_EBS_InputSignals.pne_brk_Trailer02Axle4_BrakingForce_at8p5bar_0 [-]"; p212 "pne_brk_Trailer02Axle4_torque_sns (init) export=true name=pne_brk_Trailer02Axle4_torque_sns prio=1 dataSetName=std dataClassType=initIO dataClassName=initIO unit=kg description='pne_brk_Trailer02Axle4_torque_sns': IO_EBS_InputSignals.pne_brk_Trailer02Axle4_torque_sns_0 [-]"; p213 "pne_brk_Trailer02Axle5_BrakingForce_at8p5bar [N] (init) export=true name=pne_brk_Trailer02Axle5_BrakingForce_at8p5bar prio=1 dataSetName=std dataClassType=initIO dataClassName=initIO unit=N description='pne_brk_Trailer02Axle5_BrakingForce_at8p5bar [N] (init)': IO_EBS_InputSignals.pne_brk_Trailer02Axle5_BrakingForce_at8p5bar_0 [-]"; p214 "pne_brk_Trailer02Axle5_torque_sns (init) export=true name=pne_brk_Trailer02Axle5_torque_sns prio=1 dataSetName=std dataClassType=initIO dataClassName=initIO unit=kg description='pne_brk_Trailer02Axle5_torque_sns': IO_EBS_InputSignals.pne_brk_Trailer02Axle5_torque_sns_0 [-]"; p215 "pne_brk_Trailer02Axle6_BrakingForce_at8p5bar [N] (init) export=true name=pne_brk_Trailer02Axle6_BrakingForce_at8p5bar prio=1 dataSetName=std dataClassType=initIO dataClassName=initIO unit=N description='pne_brk_Trailer02Axle6_BrakingForce_at8p5bar [N] (init)': IO_EBS_InputSignals.pne_brk_Trailer02Axle6_BrakingForce_at8p5bar_0 [-]"; p216 "pne_brk_Trailer02Axle6_torque_sns (init) export=true name=pne_brk_Trailer02Axle6_torque_sns prio=1 dataSetName=std dataClassType=initIO dataClassName=initIO unit=kg description='pne_brk_Trailer02Axle6_torque_sns': IO_EBS_InputSignals.pne_brk_Trailer02Axle6_torque_sns_0 [-]"; p217 "pne_brk_TrailerAxle1_BrakingForce_at8p5bar [N] (init) export=true name=pne_brk_TrailerAxle1_BrakingForce_at8p5bar prio=1 dataSetName=std dataClassType=initIO dataClassName=initIO unit=N description='pne_brk_TrailerAxle1_BrakingForce_at8p5bar [N] (init)': IO_EBS_InputSignals.pne_brk_TrailerAxle1_BrakingForce_at8p5bar_0 [-]"; p218 "pne_brk_TrailerAxle1_torque_sns export=true name=pne_brk_TrailerAxle1_torque_sns prio=1 dataSetName=std dataClassType=initIO dataClassName=initIO unit='-' description='pne_brk_TrailerAxle1_torque_sns': IO_EBS_InputSignals.pne_brk_TrailerAxle1_torque_sns_0 [-]"; p219 "pne_brk_TrailerAxle2_BrakingForce_at8p5bar [N] (init) export=true name=pne_brk_TrailerAxle2_BrakingForce_at8p5bar prio=1 dataSetName=std dataClassType=initIO dataClassName=initIO unit=N description='pne_brk_TrailerAxle2_BrakingForce_at8p5bar [N] (init)': IO_EBS_InputSignals.pne_brk_TrailerAxle2_BrakingForce_at8p5bar_0 [-]"; p220 "pne_brk_TrailerAxle2_torque_sns export=true name=pne_brk_TrailerAxle2_torque_sns prio=1 dataSetName=std dataClassType=initIO dataClassName=initIO unit='-' description='pne_brk_TrailerAxle2_torque_sns': IO_EBS_InputSignals.pne_brk_TrailerAxle2_torque_sns_0 [-]"; p221 "pne_brk_TrailerAxle3_BrakingForce_at8p5bar [N] (init) export=true name=pne_brk_TrailerAxle3_BrakingForce_at8p5bar prio=1 dataSetName=std dataClassType=initIO dataClassName=initIO unit=N description='pne_brk_TrailerAxle3_BrakingForce_at8p5bar [N] (init)': IO_EBS_InputSignals.pne_brk_TrailerAxle3_BrakingForce_at8p5bar_0 [-]"; p222 "pne_brk_TrailerAxle3_torque_sns export=true name=pne_brk_TrailerAxle3_torque_sns prio=1 dataSetName=std dataClassType=initIO dataClassName=initIO unit='-' description='pne_brk_TrailerAxle3_torque_sns': IO_EBS_InputSignals.pne_brk_TrailerAxle3_torque_sns_0 [-]"; p223 "PwrVehWeight_Cval (init) export=true name=PwrVehWeight_Cval prio=1 dataSetName=std dataClassType=initIO dataClassName=initIO unit=kg description='PwrVehWeight_Cval': IO_EBS_InputSignals.PwrVehWeight_Cval_0 [-]"; p224 "Retarder Percent Torque Actual 2 Current value from CPC3 export=true name=RetPctTrqActl2_Cval_CPC3 prio=1 dataSetName=std dataClassType=initIO dataClassName=initIO unit='-' description='Retarder Percent Torque Actual 2 Current value from CPC3': IO_EBS_InputSignals.RetPctTrqActl2_Cval_CPC3_0 [-]"; p225 "Retarder Reference Torque Value export=true name=RetRefTrq_Cval prio=1 dataSetName=std dataClassType=initIO dataClassName=initIO unit='-' description='Retarder Reference Torque Value': IO_EBS_InputSignals.RetRefTrq_Cval_0 [-]"; p226 "Road Curvature Current value, 65535 SNA; export=true name=RoadCurv_Cval prio=1 dataSetName=std dataClassType=initIO dataClassName=initIO unit='1/km' description='Road Curvature Current value, 65535 SNA;': IO_EBS_InputSignals.RoadCurv_Cval_0 [-]"; p227 "ROP_BrkCtrlActv2_Stat export=true name=ROP_BrkCtrlActv2_Stat prio=1 dataSetName=std dataClassType=initIO dataClassName=initIO unit='-' description='ROP_BrkCtrlActv2_Stat': IO_EBS_InputSignals.ROP_BrkCtrlActv2_Stat_0 [-]"; p228 "ROP_EngCtrlActv2_Stat export=true name=ROP_EngCtrlActv2_Stat prio=1 dataSetName=std dataClassType=initIO dataClassName=initIO unit='-' description='ROP_EngCtrlActv2_Stat': IO_EBS_InputSignals.ROP_EngCtrlActv2_Stat_0 [-]"; p229 "sAccel_X_Cval_SBSP export=true name=sAccel_X_Cval_SBSP prio=1 dataSetName=std dataClassType=initIO dataClassName=initIO unit='m/s^2' description='sAccel_X_Cval_SBSP': IO_EBS_InputSignals.sAccel_X_Cval_SBSP_0 [-]"; p230 "sAccel_Y_Cval_SBSP export=true name=sAccel_Y_Cval_SBSP prio=1 dataSetName=std dataClassType=initIO dataClassName=initIO unit='m/s^2' description='sAccel_Y_Cval_SBSP': IO_EBS_InputSignals.sAccel_Y_Cval_SBSP_0 [-]"; p231 "sAddInfoVehSped_Cval_SBSP export=true name=sAddInfoVehSped_Cval_SBSP prio=1 dataSetName=std dataClassType=initIO dataClassName=initIO unit='-' description='sAddInfoVehSped_Cval_SBSP': IO_EBS_InputSignals.sAddInfoVehSped_Cval_SBSP_0 [-]"; p232 "sBrkPdlPosn3_Cval_SBSP export=true name=sBrkPdlPosn3_Cval_SBSP prio=1 dataSetName=std dataClassType=initIO dataClassName=initIO unit='%' description='sBrkPdlPosn3_Cval_SBSP': IO_EBS_InputSignals.sBrkPdlPosn3_Cval_SBSP_0 [-]"; p233 "sBS_Brk_Cval_SBSP export=true name=sBS_Brk_Cval_SBSP prio=1 dataSetName=std dataClassType=initIO dataClassName=initIO unit='%' description='sBS_Brk_Cval_SBSP': IO_EBS_InputSignals.sBS_Brk_Cval_SBSP_0 [-]"; p234 "sBS_CS_Acc_Stat_SBSP export=true name=sBS_CS_Acc_Stat_SBSP prio=1 dataSetName=std dataClassType=initIO dataClassName=initIO unit='-' description='sBS_CS_Acc_Stat_SBSP': IO_EBS_InputSignals.sBS_CS_Acc_Stat_SBSP_0 [-]"; p235 "sBS_CS_RqPerf2_Stat_SBSP export=true name=sBS_CS_RqPerf2_Stat_SBSP prio=1 dataSetName=std dataClassType=initIO dataClassName=initIO unit='-' description='sBS_CS_RqPerf2_Stat_SBSP': IO_EBS_InputSignals.sBS_CS_RqPerf2_Stat_SBSP_0 [-]"; p236 "sBS_CS_RqPerf_Stat_SBSP export=true name=sBS_CS_RqPerf_Stat_SBSP prio=1 dataSetName=std dataClassType=initIO dataClassName=initIO unit='-' description='sBS_CS_RqPerf_Stat_SBSP': IO_EBS_InputSignals.sBS_CS_RqPerf_Stat_SBSP_0 [-]"; p237 "sBS_CSCPC_Acc_Stat_SBSP export=true name=sBS_CSCPC_Acc_Stat_SBSP prio=1 dataSetName=std dataClassType=initIO dataClassName=initIO unit='-' description='sBS_CSCPC_Acc_Stat_SBSP': IO_EBS_InputSignals.sBS_CSCPC_Acc_Stat_SBSP_0 [-]"; p238 "sBS_HB_Acc_Stat_SBSP export=true name=sBS_HB_Acc_Stat_SBSP prio=1 dataSetName=std dataClassType=initIO dataClassName=initIO unit='-' description='sBS_HB_Acc_Stat_SBSP': IO_EBS_InputSignals.sBS_HB_Acc_Stat_SBSP_0 [-]"; p239 "sBS_HB_RqPerf_Stat_SBSP export=true name=sBS_HB_RqPerf_Stat_SBSP prio=1 dataSetName=std dataClassType=initIO dataClassName=initIO unit='-' description='sBS_HB_RqPerf_Stat_SBSP': IO_EBS_InputSignals.sBS_HB_RqPerf_Stat_SBSP_0 [-]"; p240 "sBS_HBCPC_Acc_Stat_SBSP export=true name=sBS_HBCPC_Acc_Stat_SBSP prio=1 dataSetName=std dataClassType=initIO dataClassName=initIO unit='-' description='sBS_HBCPC_Acc_Stat_SBSP': IO_EBS_InputSignals.sBS_HBCPC_Acc_Stat_SBSP_0 [-]"; p241 "sBS_HBCPC_RqPerf_Stat_SBSP export=true name=sBS_HBCPC_RqPerf_Stat_SBSP prio=1 dataSetName=std dataClassType=initIO dataClassName=initIO unit='-' description='sBS_HBCPC_RqPerf_Stat_SBSP': IO_EBS_InputSignals.sBS_HBCPC_RqPerf_Stat_SBSP_0 [-]"; p242 "sBS_SS_Acc_Stat_SBSP export=true name=sBS_SS_Acc_Stat_SBSP prio=1 dataSetName=std dataClassType=initIO dataClassName=initIO unit='-' description='sBS_SS_Acc_Stat_SBSP': IO_EBS_InputSignals.sBS_SS_Acc_Stat_SBSP_0 [-]"; p243 "sBS_SS_RqPerf_Stat_SBSP export=true name=sBS_SS_RqPerf_Stat_SBSP prio=1 dataSetName=std dataClassType=initIO dataClassName=initIO unit='-' description='sBS_SS_RqPerf_Stat_SBSP': IO_EBS_InputSignals.sBS_SS_RqPerf_Stat_SBSP_0 [-]"; p244 "sConfLatAccel_SBSP export=true name=sConfLatAccel_SBSP prio=1 dataSetName=std dataClassType=initIO dataClassName=initIO unit='%' description='sConfLatAccel_SBSP': IO_EBS_InputSignals.sConfLatAccel_SBSP_0 [-]"; p245 "sConfLgtAccel_SBSP export=true name=sConfLgtAccel_SBSP prio=1 dataSetName=std dataClassType=initIO dataClassName=initIO unit='%' description='sConfLgtAccel_SBSP': IO_EBS_InputSignals.sConfLgtAccel_SBSP_0 [-]"; p246 "sConfYawRate_SBSP export=true name=sConfYawRate_SBSP prio=1 dataSetName=std dataClassType=initIO dataClassName=initIO unit='%' description='sConfYawRate_SBSP': IO_EBS_InputSignals.sConfYawRate_SBSP_0 [-]"; p247 "sEBS_BrkSw2_Rq_SBSP export=true name=sEBS_BrkSw2_Rq_SBSP prio=1 dataSetName=std dataClassType=initIO dataClassName=initIO unit='-' description='sEBS_BrkSw2_Rq_SBSP': IO_EBS_InputSignals.sEBS_BrkSw2_Rq_SBSP_0 [-]"; p248 "Full Braking Allowed state export=true name=sFullBrkAllow_Stat_SBSP prio=1 dataSetName=std dataClassType=initIO dataClassName=initIO unit='-' description='Full Braking Allowed state': IO_EBS_InputSignals.sFullBrkAllow_Stat_SBSP_0 [-]"; p249 "wheel speed of the truck front left wheel [km/h] export=true name=SpdFtAxleLtWhl_Cval prio=1 dataSetName=std dataClassType=initIO dataClassName=initIO unit='km/h' description='wheel speed of the truck front left wheel [km/h]': IO_EBS_InputSignals.SpdFtAxleLtWhl_Cval_0 [-]"; p250 "wheel speed of the truck front left wheel [km/h] export=true name=SpdFtAxleLtWhl_Cval_SBSP prio=1 dataSetName=std dataClassType=initIO dataClassName=initIO unit='km/h' description='wheel speed of the truck front left wheel [km/h]': IO_EBS_InputSignals.SpdFtAxleLtWhl_Cval_SBSP_0 [-]"; p251 "wheel speed of the truck front right wheel [km/h] export=true name=SpdFtAxleRtWhl_Cval prio=1 dataSetName=std dataClassType=initIO dataClassName=initIO unit='km/h' description='wheel speed of the truck front right wheel [km/h]': IO_EBS_InputSignals.SpdFtAxleRtWhl_Cval_0 [-]"; p252 "wheel speed of the truck front right wheel [km/h] export=true name=SpdFtAxleRtWhl_Cval_SBSP prio=1 dataSetName=std dataClassType=initIO dataClassName=initIO unit='km/h' description='wheel speed of the truck front right wheel [km/h]': IO_EBS_InputSignals.SpdFtAxleRtWhl_Cval_SBSP_0 [-]"; p253 "wheel speed of the truck rear left wheel [km/h] export=true name=SpdR_AxleLtWhl_Cval prio=1 dataSetName=std dataClassType=initIO dataClassName=initIO unit='km/h' description='wheel speed of the truck rear left wheel [km/h]': IO_EBS_InputSignals.SpdR_AxleLtWhl_Cval_0 [-]"; p254 "wheel speed of the truck rear left wheel [km/h] export=true name=SpdR_AxleLtWhl_Cval_SBSP prio=1 dataSetName=std dataClassType=initIO dataClassName=initIO unit='km/h' description='wheel speed of the truck rear left wheel [km/h]': IO_EBS_InputSignals.SpdR_AxleLtWhl_Cval_SBSP_0 [-]"; p255 "wheel speed of the truck rear right wheel [km/h] export=true name=SpdR_AxleRtWhl_Cval prio=1 dataSetName=std dataClassType=initIO dataClassName=initIO unit='km/h' description='wheel speed of the truck rear right wheel [km/h]': IO_EBS_InputSignals.SpdR_AxleRtWhl_Cval_0 [-]"; p256 "wheel speed of the truck rear right wheel [km/h] export=true name=SpdR_AxleRtWhl_Cval_SBSP prio=1 dataSetName=std dataClassType=initIO dataClassName=initIO unit='km/h' description='wheel speed of the truck rear right wheel [km/h]': IO_EBS_InputSignals.SpdR_AxleRtWhl_Cval_SBSP_0 [-]"; p257 "SrcAdrBrkCtrlDev_Cval export=true name=SrcAdrBrkCtrlDev_Cval prio=1 dataSetName=std dataClassType=initIO dataClassName=initIO unit='-' description='SrcAdrBrkCtrlDev_Cval': IO_EBS_InputSignals.SrcAdrBrkCtrlDev_Cval_0 [-]"; p258 "SrcAdrBrkCtrlDev_Cval_SBSP export=true name=SrcAdrBrkCtrlDev_Cval_SBSP prio=1 dataSetName=std dataClassType=initIO dataClassName=initIO unit='-' description='SrcAdrBrkCtrlDev_Cval_SBSP': IO_EBS_InputSignals.SrcAdrBrkCtrlDev_Cval_SBSP_0 [-]"; p259 "sSpdFtAxleLtWhl_Cval_SBSP export=true name=sSpdFtAxleLtWhl_Cval_SBSP prio=1 dataSetName=std dataClassType=initIO dataClassName=initIO unit='km/h' description='sSpdFtAxleLtWhl_Cval_SBSP': IO_EBS_InputSignals.sSpdFtAxleLtWhl_Cval_SBSP_0 [-]"; p260 "sSpdFtAxleRtWhl_Cval_SBSP export=true name=sSpdFtAxleRtWhl_Cval_SBSP prio=1 dataSetName=std dataClassType=initIO dataClassName=initIO unit='km/h' description='sSpdFtAxleRtWhl_Cval_SBSP': IO_EBS_InputSignals.sSpdFtAxleRtWhl_Cval_SBSP_0 [-]"; p261 "sSpdR_AxleLtWhl_Cval_SBSP export=true name=sSpdR_AxleLtWhl_Cval_SBSP prio=1 dataSetName=std dataClassType=initIO dataClassName=initIO unit='km/h' description='sSpdR_AxleLtWhl_Cval_SBSP': IO_EBS_InputSignals.sSpdR_AxleLtWhl_Cval_SBSP_0 [-]"; p262 "sSpdR_AxleRtWhl_Cval_SBSP export=true name=sSpdR_AxleRtWhl_Cval_SBSP prio=1 dataSetName=std dataClassType=initIO dataClassName=initIO unit='km/h' description='sSpdR_AxleRtWhl_Cval_SBSP': IO_EBS_InputSignals.sSpdR_AxleRtWhl_Cval_SBSP_0 [-]"; p263 "sSrcAdrBrkCtrlDev_Cval_SBSP export=true name=sSrcAdrBrkCtrlDev_Cval_SBSP prio=1 dataSetName=std dataClassType=initIO dataClassName=initIO unit='-' description='sSrcAdrBrkCtrlDev_Cval_SBSP': IO_EBS_InputSignals.sSrcAdrBrkCtrlDev_Cval_SBSP_0 [-]"; p264 "sStandstill_Dtct_Stat_SBSP export=true name=sStandstill_Dtct_Stat_SBSP prio=1 dataSetName=std dataClassType=initIO dataClassName=initIO unit='-' description='sStandstill_Dtct_Stat_SBSP': IO_EBS_InputSignals.sStandstill_Dtct_Stat_SBSP_0 [-]"; p265 "Standstill_Dtct_Stat_SBSP (init) export=true name=Standstill_Dtct_Stat_SBSP prio=1 dataSetName=std dataClassType=initIO dataClassName=initIO unit='-' description='Standstill_Dtct_Stat_SBSP': IO_EBS_InputSignals.Standstill_Dtct_Stat_SBSP_0 [-]"; p266 "sTrlrAbsOper_Stat export=true name=sTrlrAbsOper_Stat prio=1 dataSetName=std dataClassType=initIO dataClassName=initIO unit='-' description='sTrlrAbsOper_Stat': IO_EBS_InputSignals.sTrlrAbsOper_Stat_0 [-]"; p267 "sTrlrEstm_Stat_SBSP export=true name=sTrlrEstm_Stat_SBSP prio=1 dataSetName=std dataClassType=initIO dataClassName=initIO unit='-' description='sTrlrEstm_Stat_SBSP': IO_EBS_InputSignals.sTrlrEstm_Stat_SBSP_0 [-]"; p268 "sVehSpd_Cval_SBSP export=true name=sVehSpd_Cval_SBSP prio=1 dataSetName=std dataClassType=initIO dataClassName=initIO unit='km/h' description='sVehSpd_Cval_SBSP': IO_EBS_InputSignals.sVehSpd_Cval_SBSP_0 [-]"; p269 "sXBR_AccelLim_Stat_SBSP export=true name=sXBR_AccelLim_Stat_SBSP prio=1 dataSetName=std dataClassType=initIO dataClassName=initIO unit='m/s^2' description='sXBR_AccelLim_Stat_SBSP': IO_EBS_InputSignals.sXBR_AccelLim_Stat_SBSP_0 [-]"; p270 "sXBR_ActCtrl_Stat_SBSP export=true name=sXBR_ActCtrl_Stat_SBSP prio=1 dataSetName=std dataClassType=initIO dataClassName=initIO unit='-' description='sXBR_ActCtrl_Stat_SBSP': IO_EBS_InputSignals.sXBR_ActCtrl_Stat_SBSP_0 [-]"; p271 "sXBR_Sys_Stat_SBSP export=true name=sXBR_Sys_Stat_SBSP prio=1 dataSetName=std dataClassType=initIO dataClassName=initIO unit='-' description='sXBR_Sys_Stat_SBSP': IO_EBS_InputSignals.sXBR_Sys_Stat_SBSP_0 [-]"; p272 "sYawRateCorr_Cval_SBSP export=true name=sYawRateCorr_Cval_SBSP prio=1 dataSetName=std dataClassType=initIO dataClassName=initIO unit='rad/s' description='sYawRateCorr_Cval_SBSP': IO_EBS_InputSignals.sYawRateCorr_Cval_SBSP_0 [-]"; p273 "TrctrAbsOper_Stat export=true name=TrctrAbsOper_Stat prio=1 dataSetName=std dataClassType=initIO dataClassName=initIO unit='-' description='TrctrAbsOper_Stat': IO_EBS_InputSignals.TrctrAbsOper_Stat_0 [-]"; p274 "TrlrAbsOper_Stat (init) Trailer Estimation Current state BS 0-OFF, 1-ABS_SIMUL, 2-FULL, 3-SNA export=true name=TrlrAbsOper_Stat prio=1 dataSetName=std dataClassType=initIO dataClassName=initIO unit='-' description='Trailer Estimation Current state BS 0-OFF, 1-ABS_SIMUL, 2-FULL, 3-SNA': IO_EBS_InputSignals.TrlrAbsOper_Stat_0 [-]"; p275 "TrlrEstm_Stat_SBSP (init) export=true name=TrlrEstm_Stat_SBSP prio=1 dataSetName=std dataClassType=initIO dataClassName=initIO unit='-' description='TrlrEstm_Stat_SBSP': IO_EBS_InputSignals.TrlrEstm_Stat_SBSP_0 [-]"; p276 "TrqConv_Cval_PT export=true name=TrqConv_Cval_PT prio=1 dataSetName=std dataClassType=initIO dataClassName=initIO unit='-' description='TrqConv_Cval_PT': IO_EBS_InputSignals.TrqConv_Cval_PT_0 [-]"; p277 "Gearbox InputShaft Speed RPM Current value from CPC export=true name=TxInShaftSpd_Cval_CPC prio=1 dataSetName=std dataClassType=initIO dataClassName=initIO unit='-' description='Gearbox InputShaft Speed RPM Current value from CPC': IO_EBS_InputSignals.TxInShaftSpd_Cval_CPC_0 [-]"; p278 "Tyre Correction Value Front Axel left, 255 SNA; export=true name=TyreCorrLtFA_Cval prio=1 dataSetName=std dataClassType=initIO dataClassName=initIO unit='%' description='Tyre Correction Value Front Axel left, 255 SNA;': IO_EBS_InputSignals.TyreCorrLtFA_Cval_0 [-]"; p279 "Tyre Correction Value Rear Axel left, 255 SNA; export=true name=TyreCorrLtRA_Cval prio=1 dataSetName=std dataClassType=initIO dataClassName=initIO unit='%' description='Tyre Correction Value Rear Axel left, 255 SNA;': IO_EBS_InputSignals.TyreCorrLtRA_Cval_0 [-]"; p280 "Tyre Correction Value Front Axel Right, 255 SNA; export=true name=TyreCorrRtFA_Cval prio=1 dataSetName=std dataClassType=initIO dataClassName=initIO unit='%' description='Tyre Correction Value Front Axel Right, 255 SNA;': IO_EBS_InputSignals.TyreCorrRtFA_Cval_0 [-]"; p281 "Tyre Correction Value Rear Axel right, 255 SNA; export=true name=TyreCorrRtRA_Cval prio=1 dataSetName=std dataClassType=initIO dataClassName=initIO unit='%' description='Tyre Correction Value Rear Axel right, 255 SNA;': IO_EBS_InputSignals.TyreCorrRtRA_Cval_0 [-]"; p282 "Tyre Rolling Circumference Front Axel, 255 SNA; export=true name=TyreRollCircumFA_Cval prio=1 dataSetName=std dataClassType=initIO dataClassName=initIO unit='mm' description='Tyre Rolling Circumference Front Axel, 255 SNA;': IO_EBS_InputSignals.TyreRollCircumFA_Cval_0 [-]"; p283 "Tyre Rolling Circumference Rear Axel, 255 SNA; export=true name=TyreRollCircumRA_Cval prio=1 dataSetName=std dataClassType=initIO dataClassName=initIO unit='mm' description='Tyre Rolling Circumference Rear Axel, 255 SNA;': IO_EBS_InputSignals.TyreRollCircumRA_Cval_0 [-]"; p284 "Trailer Velocity export=true name=VehSpd1_Cval_Trlr prio=1 dataSetName=std dataClassType=initIO dataClassName=initIO unit='-' description='Trailer Velocity': IO_EBS_InputSignals.VehSpd1_Cval_Trlr_0 [-]"; p285 "speed of the truck [km/h] export=true name=VehSpd_Cval_BS prio=1 dataSetName=std dataClassType=initIO dataClassName=initIO unit='km/h' description='speed of the truck [km/h]': IO_EBS_InputSignals.VehSpd_Cval_BS_0 [-]"; p286 "VehSpd_Cval_SBSP (init) export=true name=VehSpd_Cval_SBSP prio=1 dataSetName=std dataClassType=initIO dataClassName=initIO unit='km/h' description='VehSpd_Cval_SBSP': IO_EBS_InputSignals.VehSpd_Cval_SBSP_0 [-]"; p287 "XBR_AccelLim_Stat_BS export=true name=XBR_AccelLim_Stat_BS prio=1 dataSetName=std dataClassType=initIO dataClassName=initIO unit=m/s^2 description='XBR_AccelLim_Stat_BS': IO_EBS_InputSignals.XBR_AccelLim_Stat_BS_0 [-]"; p288 "XBR_AccelLim_Stat_SBSP export=true name=XBR_AccelLim_Stat_SBSP prio=1 dataSetName=std dataClassType=initIO dataClassName=initIO unit=m/s^2 description='XBR_AccelLim_Stat_SBSP': IO_EBS_InputSignals.XBR_AccelLim_Stat_SBSP_0 [-]"; p289 "XBR_ActCtrl_Stat_SBSP export=true name=XBR_ActCtrl_Stat_SBSP prio=1 dataSetName=std dataClassType=initIO dataClassName=initIO unit='-' description='XBR_ActCtrl_Stat_SBSP': IO_EBS_InputSignals.XBR_ActCtrl_Stat_SBSP_0 [-]"; p290 "XBR_CtrlMode_Stat_CPC5ce export=true name=XBR_CtrlMode_Stat_CPC5ce prio=1 dataSetName=std dataClassType=initIO dataClassName=initIO unit='-' description='XBR_CtrlMode_Stat_CPC5ce': IO_EBS_InputSignals.XBR_CtrlMode_Stat_CPC5ce_0 [-]"; p291 "XBR_CtrlMode_Stat_VRDU export=true name=XBR_CtrlMode_Stat_VRDU prio=1 dataSetName=std dataClassType=initIO dataClassName=initIO unit='-' description='XBR_CtrlMode_Stat_VRDU': IO_EBS_InputSignals.XBR_CtrlMode_Stat_VRDU_0 [-]"; p292 "XBR_EBI_Stat_VRDU export=true name=XBR_EBI_Stat_VRDU prio=1 dataSetName=std dataClassType=initIO dataClassName=initIO unit='-' description='XBR_EBI_Stat_VRDU': IO_EBS_InputSignals.XBR_EBI_Stat_VRDU_0 [-]"; p293 "XBR_Prio_Stat_CPC5ce export=true name=XBR_Prio_Stat_CPC5ce prio=1 dataSetName=std dataClassType=initIO dataClassName=initIO unit='-' description='XBR_Prio_Stat_CPC5ce': IO_EBS_InputSignals.XBR_Prio_Stat_CPC5ce_0 [-]"; p294 "XBR_Prio_Stat_VRDU export=true name=XBR_Prio_Stat_VRDU prio=1 dataSetName=std dataClassType=initIO dataClassName=initIO unit='-' description='XBR_Prio_Stat_VRDU': IO_EBS_InputSignals.XBR_Prio_Stat_VRDU_0 [-]"; p295 "XBR_Sys_Stat_SBSP export=true name=XBR_Sys_Stat_SBSP prio=1 dataSetName=std dataClassType=initIO dataClassName=initIO unit='-' description='XBR_Sys_Stat_SBSP': IO_EBS_InputSignals.XBR_Sys_Stat_SBSP_0 [-]"; p296 "YawRateCorr_Cval_SBSP export=true name=YawRateCorr_Cval_SBSP prio=1 dataSetName=std dataClassType=initIO dataClassName=initIO unit='rad/s' description='YawRateCorr_Cval_SBSP': IO_EBS_InputSignals.YawRateCorr_Cval_SBSP_0 [-]"; p297 "YC_BrkCtrlActv2_Stat export=true name=YC_BrkCtrlActv2_Stat prio=1 dataSetName=std dataClassType=initIO dataClassName=initIO unit='-' description='YC_BrkCtrlActv2_Stat': IO_EBS_InputSignals.YC_BrkCtrlActv2_Stat_0 [-]"; p298 "YC_EngCtrlActv2_Stat export=true name=YC_EngCtrlActv2_Stat prio=1 dataSetName=std dataClassType=initIO dataClassName=initIO unit='-' description='YC_EngCtrlActv2_Stat': IO_EBS_InputSignals.YC_EngCtrlActv2_Stat_0 [-]"; p299 "Nominal InputShaft Displacement [-] export=true name=zSoll_dx_xAxis_nom prio=1 dataSetName=ebs_dummy dataClassType=main dataClassName=main  unit='-' description='Nominal InputShaft Displacement [-]': BWG.zSoll_dx_xAxis_nom [-]"; p300 "Nominal InputShaft Displacement [-] export=true name=zSoll_dx_yAxis_nom prio=1 dataSetName=ebs_dummy dataClassType=main dataClassName=main  unit='-' description='Nominal Deceleration Set Value [-]': BWG.zSoll_dx_yAxis_nom [-]"; p301 "Axle Loads Trailer export=true name=axleLoadTrailer02_kg prio=1 dataSetName=veh_dummy dataClassType=veh dataClassName=veh unit=kg description='Axle Loads Trailer02': eBS_veh_Param.axleLoadTrailer02_kg [-]"; p302 "Axle Loads Trailer export=true name=axleLoadTrailer_kg prio=1 dataSetName=veh_dummy dataClassType=veh dataClassName=veh unit=kg description='Axle Loads Trailer': eBS_veh_Param.axleLoadTrailer_kg [-]"; p303 "Axle Loads Vehicle export=true name=axleLoadVehicle_kg prio=1 dataSetName=veh_dummy dataClassType=veh dataClassName=veh unit=kg description='Axle Loads Vehicle': eBS_veh_Param.axleLoadVehicle_kg [-]"; p304 "Brake Circuit Configuration [A1, A2, A3, A4] (0-Dummy, 1-Front, 2-Rear, 3-Middle(Bus)) export=true name=brkCircuit prio=1 dataSetName=veh_dummy dataClassType=veh dataClassName=veh unit='-' description='Brake Circuit Configuration [A1, A2, A3, A4] (0-Dummy, 1-Front, 2-Rear, 3-Middle(Bus))': eBS_veh_Param.brkCircuit [-]"; p305 "Trailer Control Active / Trailer can brake {flag, x1, x2, x3, x4, x5, y1, y2, y3, y4, y5} (flag: 0 - no, 1- yes ALB lower limit, 2- yes ALB normal, 3- yes ALB upper limit , 4 - yes without ALB, 5 - with characteristics {{x1 ...x5},{y1...y5}) export=true name=flagTrailer02ControlActive prio=1 dataSetName=veh_dummy dataClassType=veh dataClassName=veh unit='-' description='Trailer Control Active / Trailer can brake {flag, x1, x2, x3, x4, x5, y1, y2, y3, y4, y5} (flag: 0 - no, 1- yes ALB lower limit, 2- yes ALB normal, 3- yes ALB upper limit , 4 - yes without ALB, 5 - with characteristics {{x1 ...x5},{y1...y5})': eBS_veh_Param.flagTrailer02ControlActive [-]"; p306 "Trailer Control Active / Trailer can brake {flag, x1, x2, x3, x4, x5, y1, y2, y3, y4, y5} (flag: 0 - no, 1- yes ALB lower limit, 2- yes ALB normal, 3- yes ALB upper limit , 4 - yes without ALB, 5 - with characteristics {{x1 ...x5},{y1...y5}) export=true name=flagTrailerControlActive prio=1 dataSetName=veh_dummy dataClassType=veh dataClassName=veh unit='-' description='Trailer Control Active / Trailer can brake {flag, x1, x2, x3, x4, x5, y1, y2, y3, y4, y5} (flag: 0 - no, 1- yes ALB lower limit, 2- yes ALB normal, 3- yes ALB upper limit , 4 - yes without ALB, 5 - with characteristics {{x1 ...x5},{y1...y5})': eBS_veh_Param.flagTrailerControlActive [-]"; p307 "pAppCyl Tractor Axles [A1, A2, A3, A4] [bar] export=true name=pAppCyl_Tractor prio=1 dataSetName=veh_dummy dataClassType=veh dataClassName=veh unit='bar' description='pAppCyl Tractor Axles [A1, A2, A3, A4] [bar]': eBS_veh_Param.pAppCyl_Tractor [-]"; p308 "pAppCyl Trailer Axles [TA1, TA2, TA3] [bar] export=true name=pAppCyl_Trailer prio=1 dataSetName=veh_dummy dataClassType=veh dataClassName=veh unit='bar' description='pAppCyl Trailer Axles [TA1, TA2, TA3] [bar]': eBS_veh_Param.pAppCyl_Trailer [-]"; p309 "application pressure of trailer axles [A1, A2, A3, A4, A5, A6] [bar] export=true name=pAppCyl_Trailer02 prio=1 dataSetName=veh_dummy dataClassType=veh dataClassName=veh unit='bar' description='application pressure of trailer axles [A1, A2, A3, A4, A5, A6]  [bar]': eBS_veh_Param.pAppCyl_Trailer02 [-]"; p310 "rdyn's of Trailer02 [A1,A2,A3, A4, A5, A6] export=true name=rdynTrailer02 prio=1 dataSetName=veh_dummy dataClassType=veh dataClassName=veh unit=mm description='Trailer02 rDyn': eBS_veh_Param.rdynTrailer02 [-]"; p311 "Vehicle Speed Sensor Axle Position {A1,A2,A3,A4} (0-false,1-true)  export=true name=speedSensorPosnVeh prio=1 dataSetName=veh_dummy dataClassType=veh dataClassName=veh unit='' description='Vehicle Speed Sensor Axle Position {A1,A2,A3,A4} (0-false,1-true)': eBS_veh_Param.speedSensorPosnVeh [-]"
